simulink model "SVM_Stepper"  (R2020b)
settings: Solver=VariableStepAuto  StartTime=0.0  StopTime=1  FixedStep=0.0001  MaxStep=0.000005  RelTol=1e-3
values from neighbouring files (symbols this model uses):
  b = 0.05    [system_parameters.m]
  J = 48e-6    (= 4.8e-05)    [system_parameters.m]
  K_t = T_hold/I_rms    (= 0.575)    [system_parameters.m]
  L = 2e-3    (= 0.002)    [system_parameters.m]
  p = 50    [system_parameters.m]
  R = 0.5    [system_parameters.m]
  T_dm = 0.068    [system_parameters.m]
  T_load = 5.06e-3    (= 0.00506)    [system_parameters.m]
  U = 24    [system_parameters.m]
undefined symbols (not defined in the file or in its folder): Down, Up
libraries: fl_lib x90, ee_lib x55, eePwmGenerator x37, nesl_utility x33, dspsrcs4 x18, pid_lib x6, powerlib x4, eeDcCurrentController x1, eePmsmTorqueEstimator x1, simulink x1, eeQuadratureDecoder x1
(part 1 of 2)
settings Model: Creator=ginoa  LastModifiedBy=ginoa

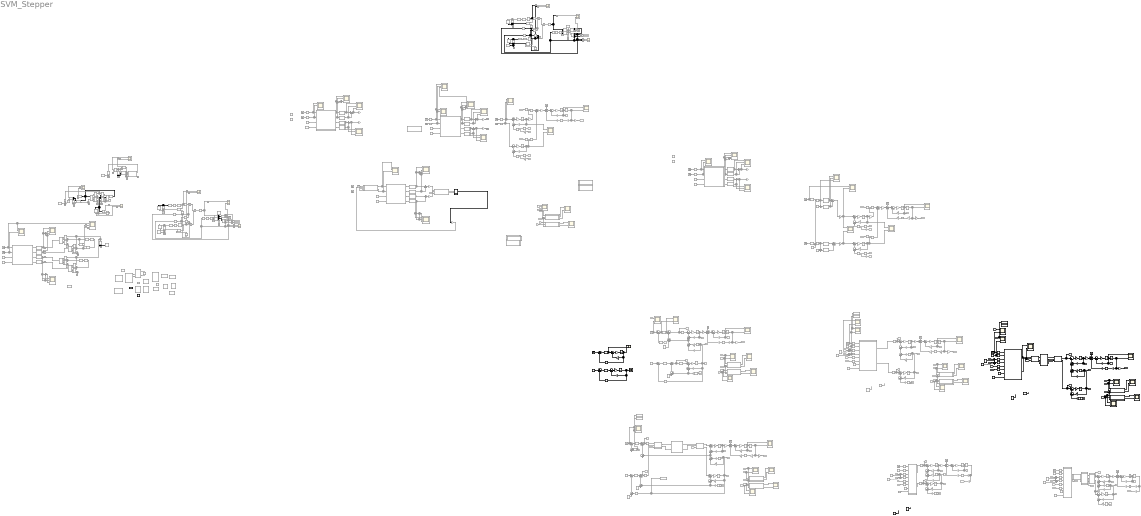
== system SVM_Stepper ==
  note: Load Torque
  note: Load Torque
  note: i_q
  note: i_d
  note: i_d
  note: i_q
  note: i_q
  note: i_d
  note: i_q
  note: i_d
  note: i_q
  note: i_d
  note: i_q
  note: i_d
  note: i_q
  note: i_d
  CMOS NOT : ee_lib/Integrated Circuits/Logic/CMOS NOT  Commented=on  V_IL=2 V  V_IH=3 V  C_IN=5 pF  output_type=1  V_OL=0 V  V_OH=5 V  V_CC=5 V  V_meas=5 V  R_OUT=25 Ohm  R_OH=[25, 250] Ohm  I_OH=63 mA  R_OL=[30, 800] Ohm  I_OL=-45 mA  Delay=25 ns  Ron=5 Ohm  Vf=0.6 V  output_state=1
      settings: SourceProductBaseCode=PS  InternalSimscapePortConfiguration="{\"Bottom\":[],\"Left\":[{\"id\":\"A\",\"label\":\"\",\"type\":\"foundation.electrical.electrical\"}],\"Right\":[{\"id\":\"J\",\"label\":\"\",\"type\":\"foundation.electrical.electrical\"}],\"Top\":[]}"
  Constant{,2,9,13,20,27,30} (7 alike) : Constant  Commented=on  Value=24
  Constant1 : Constant  Commented=on  Value=50e-6
  Constant10 : Constant  Commented=on  Value=48
  Constant11 : Constant  Commented=on  Value=25e-6
  Constant12 : Constant  Commented=on  Value=10
  Constant14 : Constant  Commented=on
  Constant15 : Constant  Commented=on  Value=48
  Constant16 : Constant  Commented=on
  Constant{17,19,22,26,29} (5 alike) : Constant  Commented=on  Value=0
  Constant18 : Constant  Value=0
  Constant21 : Constant  Commented=on  Value=20e-6
  Constant23 : Constant  Value=0
  Constant24 : Constant  Value=24
  Constant25 : Constant  Value=50e-6
  Constant28 : Constant  Commented=on  Value=50e-6
  Constant3 : Constant  Commented=on  Value=50e-6
  Constant31 : Constant  Commented=on  Value=20e-6
  Constant4 : Constant  Commented=on  Value=100
  Constant5 : Constant  Commented=on  Value=25e-6
  Constant6 : Constant  Commented=on  Value=48
  Constant7 : Constant  Commented=on  Value=25e-6
  Constant8 : Constant  Commented=on  Value=10
  Controlled PWM Voltage : ee_lib/Integrated Circuits/Controlled PWM Voltage  Commented=on  F=20000 Hz  TD=0 s  pulse_width_offset=0 s  pulse_min=0 s  Vmin=-24 V  Vmax=24 V  Vm=5 V  pwm_or_av=1  event_type=1  sample_time=1e-6 s  u_min=0  u_max=1
  Controlled PWM Voltage1 : ee_lib/Integrated Circuits/Controlled PWM Voltage  Commented=on  F=10000 Hz  TD=0 us  pulse_width_offset=0 s  pulse_min=4 us  Vmin=-24 V  Vmax=24 V  Vm=18 V  pwm_or_av=1  event_type=1  sample_time=1e-6 s  u_min=0  u_max=1
  Controlled PWM Voltage2 : ee_lib/Integrated Circuits/Controlled PWM Voltage  Commented=on  F=1000 Hz  TD=0 s  pulse_width_offset=0 s  pulse_min=0 s  Vmin=0 V  Vmax=5 V  Vm=5 V  pwm_or_av=1  event_type=1  sample_time=1e-6 s  u_min=0  u_max=1
  Controlled Voltage Source{,1..3} (4 alike) : fl_lib/Electrical/Electrical Sources/Controlled Voltage Source  Commented=on
  Cos{,1..3} (4 alike) : Trigonometry  Commented=on  Operator=cos
  Current Sensor{,1..5} (6 alike) : fl_lib/Electrical/Electrical Sensors/Current Sensor  Commented=on
  DC Current Controller : eeDcCurrentController/DC Current Controller  Commented=on  Kp=1  Ki=5  Kaw=1  VoltLim=Positive and negative voltage  Ts=-1  Tsd=0.001  ActZC=off
      settings: SourceProductBaseCode=PS
  DC Voltage Source : powerlib/Electrical Sources/DC Voltage Source  Commented=on  Amplitude=100  Measurements=None
  Deadbeat Control : MATLAB Function  TreatAsAtomicUnit=on
  Deadbeat Control1 : MATLAB Function  Commented=on  TreatAsAtomicUnit=on
  Divide : Product  Commented=on  Inputs=*/
  Divide1 : Product  Commented=on  Inputs=*/
  Electrical Reference{,1..21} (22 alike) : fl_lib/Electrical/Electrical Elements/Electrical Reference  Commented=on
  FCS MPC : MATLAB Function  Commented=on  TreatAsAtomicUnit=on
  FCS MPC1 : MATLAB Function  Commented=on  TreatAsAtomicUnit=on
  From{,4,22,30,45,77,86} (7 alike) : From  Commented=on  GotoTag=i_d
  From{1..3,23,26,31,34,38,44,46,49,53,72,76,80} (15 alike) : From  Commented=on  GotoTag=i_q
  From{5,8..11,13,15..17,19,21,27,35,41,50,54..55,79,82..83,88} (21 alike) : From  Commented=on  GotoTag=theta_e
  From{12,14,18,20,24..25,32..33,40,42..43,47..48,74..75,78,87} (17 alike) : From  Commented=on  GotoTag=w_m
  From{6,28,36,51} (4 alike) : From  Commented=on  GotoTag=u_q
  From{7,29,37,52} (4 alike) : From  Commented=on  GotoTag=u_d
  Full-Bridge Converter : powerlib/Power Electronics/Full-Bridge Converter  Commented=on  ModelType=Switching devices  Ron=1e-3  Rs=1e6  Cs=inf  Vforward=[0,0]  Ron_Diode=1e-3  Rs_Diode=1e6  Cs_Diode=inf  Vf_Diode=1e-3  Rs_CurrentSource=inf
      settings: SourceProductBaseCode=PS
  Gain{1,6,22,25,31,41,44,47,57,62,74,79,87,92,114,119} (16 alike) : Gain  Commented=on  Gain=K_t
  Gain{5,10,53,61,70,78,83,91,110,118} (10 alike) : Gain  Commented=on  Gain=L*p
  Gain100 : Gain  Gain=K_t
  Gain{64..65,101,103} (4 alike) : Gain  Gain=1/L
  Gain{63,66,95,102} (4 alike) : Gain  Gain=R
  Gain104 : Gain  Gain=L*p
  Gain105 : Gain  Gain=K_t
  Gain{20,39,56,73,86,106,113} (7 alike) : Gain  Commented=on  Gain=2*p
  Gain{7,16,35,50,67,80,107} (7 alike) : Gain  Commented=on  Gain=1/J
  Gain{8,17,36,51,68,81,108} (7 alike) : Gain  Commented=on  Gain=b
  Gain{3,9,24,30,43,46,52,59,69,76,82,89,109,116} (14 alike) : Gain  Commented=on  Gain=R
  Gain{11,18,37,54,71,84,111} (7 alike) : Gain  Commented=on  Gain=p
  Gain{13,19,38,55,72,85,112} (7 alike) : Gain  Commented=on  Gain=T_dm
  Gain{2,4,23,29,42,45,58,60,75,77,88,90,115,117} (14 alike) : Gain  Commented=on  Gain=1/L
  Gain12 : Gain  Commented=on  Gain=-1
  Gain{14..15,48..49} (4 alike) : Gain  Commented=on  Gain=24
  Gain21 : Gain  Commented=on  Gain=-1
  Gain26 : Gain  Commented=on  Gain=100
  Gain27 : Gain  Commented=on  Gain=100
  Gain{28,32..34} (4 alike) : Gain  Commented=on  Gain=48
  Gain40 : Gain  Commented=on  Gain=-1
  Gain93 : Gain  Gain=1/J
  Gain94 : Gain  Gain=b
  Gain96 : Gain  Gain=L*p
  Gain97 : Gain  Gain=p
  Gain98 : Gain  Gain=T_dm
  Gain99 : Gain  Gain=2*p
  Goto{1,14,20,26,39} (5 alike) : Goto  Commented=on  GotoTag=i_d
  Goto10 : Goto  Commented=on  GotoTag=PS_omega_m
  Goto11 : Goto  Commented=on  GotoTag=PS_theta_m
  Goto{3,8,12,16,22,28,41} (7 alike) : Goto  Commented=on  GotoTag=w_m
  Goto{6,9,13,17,23,29,42} (7 alike) : Goto  Commented=on  GotoTag=theta_e
  Goto{2,15,21,27,40} (5 alike) : Goto  Commented=on  GotoTag=i_q
  Goto{7,18,24,30,43} (5 alike) : Goto  Commented=on  GotoTag=u_q
  Goto{19,25,31,38,44} (5 alike) : Goto  Commented=on  GotoTag=u_d
  Goto4 : Goto  Commented=on  GotoTag=PS_omega_m
  Goto5 : Goto  Commented=on  GotoTag=PS_theta_m
  H-Bridge : ee_lib/Semiconductors & Converters/Converters/H-Bridge  Commented=on  supply_ports=ee.enum.supply_ports.hidesupply  Venable=2.5 V  Vmax=5.0 V  Vreverse=2.5 V  Vbrake=2.5 V  Vm=12 V  pwm_or_av=ee.enum.pwm_or_av.pwm  regenerative_braking_mode=ee.enum.converters.regenerative_braking_mode.depends_on_rev  discontinuous=ee.enum.current_profile.continuous  freewheeling_mode=ee.enum.converters.freewheeling_mode.one_switch_one_diode  Ron=0.1 Ohm  Don=0.05 Ohm  Goff=1e-6 S  Rload=10 Ohm  Lload=1e-5 H  F=10 kHz  thermal_mass=100 J/K  initial_temperature=298.15 K  Ron2=0.1 Ohm  Don2=0.05 Ohm  Tmeas=298.15 K  Tmeas2=398.15 K
  H-Bridge1 : ee_lib/Semiconductors & Converters/Converters/H-Bridge  Commented=on  supply_ports=ee.enum.supply_ports.hidesupply  Venable=2.5 V  Vmax=5.0 V  Vreverse=2.5 V  Vbrake=2.5 V  Vm=12 V  pwm_or_av=ee.enum.pwm_or_av.pwm  regenerative_braking_mode=ee.enum.converters.regenerative_braking_mode.depends_on_rev  discontinuous=ee.enum.current_profile.continuous  freewheeling_mode=ee.enum.converters.freewheeling_mode.one_switch_one_diode  Ron=0.1 Ohm  Don=0.05 Ohm  Goff=1e-6 S  Rload=10 Ohm  Lload=1e-5 H  F=10 kHz  thermal_mass=100 J/K  initial_temperature=298.15 K  Ron2=0.1 Ohm  Don2=0.05 Ohm  Tmeas=298.15 K  Tmeas2=398.15 K
  H-Bridge2 : ee_lib/Semiconductors & Converters/Converters/H-Bridge  Commented=on  supply_ports=ee.enum.supply_ports.showsupply  Venable=2.5 V  Vmax=5.0 V  Vreverse=2.5 V  Vbrake=2.5 V  Vm=12 V  pwm_or_av=ee.enum.pwm_or_av.pwm  regenerative_braking_mode=ee.enum.converters.regenerative_braking_mode.depends_on_rev  discontinuous=ee.enum.current_profile.continuous  freewheeling_mode=ee.enum.converters.freewheeling_mode.one_switch_one_diode  Ron=0.05 Ohm  Don=0.05 Ohm  Goff=1e-6 S  Rload=10 Ohm  Lload=1e-5 H  F=10 kHz  thermal_mass=100 J/K  initial_temperature=298.15 K  Ron2=0.1 Ohm  Don2=0.05 Ohm  Tmeas=298.15 K  Tmeas2=398.15 K
      settings: InternalSimscapePortConfiguration="{\"Bottom\":[],\"Left\":[{\"id\":\"ENA\",\"label\":\"PWM\",\"type\":\"foundation.electrical.electrical\"},{\"id\":\"REF\",\"label\":\"REF\",\"type\":\"foundation.electrical.electrical\"},{\"id\":\"REV\",\"label\":\"REV\",\"type\":\"foundation.electrical.electrical\"},{\"id\":\"BRK\",\"label\":\"BRK\",\"type\":\"foundation.electrical.electrical\"}],\"Right\":[{\"id\":\"p1\",\"label\":\"V+\",\"type\":\"foundation.electrical.electrical\"},{\"id\":\"p2\",\"label\":\"+\",\"type\":\"foundation.electrical.electrical\"},{\"id\":\"n2\",\"label\":\"-\",\"type\":\"foundation.electrical.electrical\"},{\"id\":\"n1\",\"label\":\"V-\",\"type\":\"foundation.electrical.electrical\"}],\"Top\":[]}"
  Half-Bridge Driver{,1..5} (6 alike) : ee_lib/Semiconductors & Converters/Half-Bridge Driver  Commented=on  vHigh=15 V  vLow=0 V  parameterization=1  rHigh=2 Ohm  rLow=2 Ohm  tRise=20 ns  tFall=20 ns  cLoad=10 nF  enable_faults=0  t_fault=1 s  fault_type=1  uHighValue=0.7  uLowValue=0.3  tpLH=50 ns  tdLH=100 ns  tpHL=50 ns  tdHL=100 ns  ZonTime_specify=off  ZonTime_priority=None  ZonTime=0 s  ZoffTime_specify=off  ZoffTime_priority=None  ZoffTime=0 s  power_dissipated_high_side_specify=off  power_dissipated_high_side_priority=None  power_dissipated_high_side=0 W  power_dissipated_high_side_nominal_specify=off  power_dissipated_high_side_nominal_unit=W  power_dissipated_high_side_nominal_value=1  power_dissipated_low_side_specify=off  power_dissipated_low_side_priority=None  power_dissipated_low_side=0 W  power_dissipated_low_side_nominal_specify=off  power_dissipated_low_side_nominal_unit=W  power_dissipated_low_side_nominal_value=1  uHigh=2.0 V  uLow=0.8 V
      Half-Bridge Driver settings: SourceProductBaseCode=PS  InternalSimscapePortConfiguration="{\"Bottom\":[],\"Left\":[{\"id\":\"PWM\",\"label\":\"PWM\",\"type\":\"foundation.electrical.electrical\"},{\"id\":\"REF\",\"label\":\"REF\",\"type\":\"foundation.electrical.electrical\"}],\"Right\":[{\"id\":\"HO\",\"label\":\"HO\",\"type\":\"foundation.electrical.electrical\"},{\"id\":\"HS\",\"label\":\"HS\",\"type\":\"foundation.electrical.electrical\"},{\"id\":\"LO\",\"label\":\"LO\",\"type\":\"foundation.electrical.electrical\"},{\"id\":\"LS\",\"label\":\"LS\",\"type\":\"foundation.electrical.electrical\"}],\"Top\":[]}"
      Half-Bridge Driver1 settings: SourceProductBaseCode=PS  InternalSimscapePortConfiguration="{\"Bottom\":[],\"Left\":[{\"id\":\"PWM\",\"label\":\"PWM\",\"type\":\"foundation.electrical.electrical\"},{\"id\":\"REF\",\"label\":\"REF\",\"type\":\"foundation.electrical.electrical\"}],\"Right\":[{\"id\":\"HO\",\"label\":\"HO\",\"type\":\"foundation.electrical.electrical\"},{\"id\":\"HS\",\"label\":\"HS\",\"type\":\"foundation.electrical.electrical\"},{\"id\":\"LO\",\"label\":\"LO\",\"type\":\"foundation.electrical.electrical\"},{\"id\":\"LS\",\"label\":\"LS\",\"type\":\"foundation.electrical.electrical\"}],\"Top\":[]}"
      Half-Bridge Driver2 settings: SourceProductBaseCode=PS  InternalSimscapePortConfiguration="{\"Bottom\":[],\"Left\":[{\"id\":\"u\",\"label\":\"u\",\"type\":\"input\"}],\"Right\":[{\"id\":\"HO\",\"label\":\"HO\",\"type\":\"foundation.electrical.electrical\"},{\"id\":\"HS\",\"label\":\"HS\",\"type\":\"foundation.electrical.electrical\"},{\"id\":\"LO\",\"label\":\"LO\",\"type\":\"foundation.electrical.electrical\"},{\"id\":\"LS\",\"label\":\"LS\",\"type\":\"foundation.electrical.electrical\"}],\"Top\":[]}"
      Half-Bridge Driver3 settings: SourceProductBaseCode=PS  InternalSimscapePortConfiguration="{\"Bottom\":[],\"Left\":[{\"id\":\"u\",\"label\":\"u\",\"type\":\"input\"}],\"Right\":[{\"id\":\"HO\",\"label\":\"HO\",\"type\":\"foundation.electrical.electrical\"},{\"id\":\"HS\",\"label\":\"HS\",\"type\":\"foundation.electrical.electrical\"},{\"id\":\"LO\",\"label\":\"LO\",\"type\":\"foundation.electrical.electrical\"},{\"id\":\"LS\",\"label\":\"LS\",\"type\":\"foundation.electrical.electrical\"}],\"Top\":[]}"
      Half-Bridge Driver4 settings: SourceProductBaseCode=PS  InternalSimscapePortConfiguration="{\"Bottom\":[],\"Left\":[{\"id\":\"u\",\"label\":\"u\",\"type\":\"input\"}],\"Right\":[{\"id\":\"HO\",\"label\":\"HO\",\"type\":\"foundation.electrical.electrical\"},{\"id\":\"HS\",\"label\":\"HS\",\"type\":\"foundation.electrical.electrical\"},{\"id\":\"LO\",\"label\":\"LO\",\"type\":\"foundation.electrical.electrical\"},{\"id\":\"LS\",\"label\":\"LS\",\"type\":\"foundation.electrical.electrical\"}],\"Top\":[]}"
      Half-Bridge Driver5 settings: SourceProductBaseCode=PS  InternalSimscapePortConfiguration="{\"Bottom\":[],\"Left\":[{\"id\":\"u\",\"label\":\"u\",\"type\":\"input\"}],\"Right\":[{\"id\":\"HO\",\"label\":\"HO\",\"type\":\"foundation.electrical.electrical\"},{\"id\":\"HS\",\"label\":\"HS\",\"type\":\"foundation.electrical.electrical\"},{\"id\":\"LO\",\"label\":\"LO\",\"type\":\"foundation.electrical.electrical\"},{\"id\":\"LS\",\"label\":\"LS\",\"type\":\"foundation.electrical.electrical\"}],\"Top\":[]}"
  Ideal Rotational Motion Sensor : fl_lib/Mechanical/Mechanical Sensors/Ideal Rotational Motion Sensor  Commented=on  wrap_angle=simscape.enum.onoff.off  offset=0 rad
  Ideal Rotational Motion Sensor1 : fl_lib/Mechanical/Mechanical Sensors/Ideal Rotational Motion Sensor  Commented=on  wrap_angle=simscape.enum.onoff.off  offset=0 rad
  Ideal Semiconductor Switch{,1..11} (12 alike) : ee_lib/Semiconductors & Converters/Ideal Semiconductor Switch  Commented=on  Ron=0.001 Ohm  Goff=1e-6 1/Ohm  Vth=0.5 V  diode_param=2  diode_Vf=0.8 V  diode_Ron=0.001 Ohm  diode_Goff=1e-5 1/Ohm  diode_C=50e-9 F  diode_iRM=-235 A  diode_iF=300 A  diode_idot=-50 A/us  diode_trr_param=1  diode_trr_factor=3  diode_trr=15 us  diode_Qrr=1500 s*uA
      settings: SourceProductBaseCode=PS  InternalSimscapePortConfiguration="{\"Bottom\":[],\"Left\":[{\"id\":\"G\",\"label\":\"\",\"type\":\"foundation.electrical.electrical\"}],\"Right\":[{\"id\":\"A\",\"label\":\"a\",\"type\":\"foundation.electrical.electrical\"},{\"id\":\"K\",\"label\":\"k\",\"type\":\"foundation.electrical.electrical\"}],\"Top\":[]}"
  Ideal Torque Source{,1..5} (6 alike) : fl_lib/Mechanical/Mechanical Sources/Ideal Torque Source  Commented=on
  Incremental Shaft Encoder : ee_lib/Sensors & Transducers/Incremental Shaft Encoder  Commented=on  NPulse=2  Vm=5 V  angle0=0 deg
      settings: SourceProductBaseCode=PS  InternalSimscapePortConfiguration="{\"Bottom\":[],\"Left\":[{\"id\":\"R\",\"label\":\"R\",\"type\":\"foundation.mechanical.rotational.rotational\"},{\"id\":\"C\",\"label\":\"C\",\"type\":\"foundation.mechanical.rotational.rotational\"}],\"Right\":[{\"id\":\"A\",\"label\":\"A\",\"type\":\"foundation.electrical.electrical\"},{\"id\":\"B\",\"label\":\"B\",\"type\":\"foundation.electrical.electrical\"},{\"id\":\"Z\",\"label\":\"Z\",\"type\":\"foundation.electrical.electrical\"},{\"id\":\"GND\",\"label\":\"REF\",\"type\":\"foundation.electrical.electrical\"}],\"Top\":[]}"
  Inductor{,1..2,4..6} (6 alike) : ee_lib/Passive/Inductor  Commented=on  l=L H  L_tol=20  enable_L_tol=0  tol_distribution=1  nSigma=4  r=0 Ohm  g=1e-9 1/Ohm  enable_operating_limits=0  operating_limit_action=2  max_working_current=1 A  power_rating=1 W  enable_faults=0  fault_action=1  lambdaPercent=50  k_faulted=0.9999  turnsShort=0  openCct=0  groundShort=0  groundShortG=0 1/Ohm  tau_fault=1e-3 s  enable_temporal_fault=0  t_fault=1 s  enable_behavioral_fault=0  max_permissible_voltage=100 V  n_fail_on_voltage=1  max_permissible_current=1 A  t_fail_on_current=1 s  i_L_specify=off  i_L_priority=High  i_L=0 A  i_L_nominal_specify=off  i_L_nominal_unit=A  i_L_nominal_value=1
  Inductor3 : ee_lib/Passive/Inductor  Commented=on  l=20 mH  L_tol=20  enable_L_tol=0  tol_distribution=1  nSigma=4  r=0 Ohm  g=1e-9 1/Ohm  enable_operating_limits=0  operating_limit_action=2  max_working_current=1 A  power_rating=1 W  enable_faults=0  fault_action=1  lambdaPercent=50  k_faulted=0.9999  turnsShort=0  openCct=0  groundShort=0  groundShortG=0 1/Ohm  tau_fault=1e-3 s  enable_temporal_fault=0  t_fault=1 s  enable_behavioral_fault=0  max_permissible_voltage=100 V  n_fail_on_voltage=1  max_permissible_current=1 A  t_fail_on_current=1 s  i_L_specify=off  i_L_priority=High  i_L=0 A  i_L_nominal_specify=off  i_L_nominal_unit=A  i_L_nominal_value=1
  Inertia : fl_lib/Mechanical/Rotational Elements/Inertia  Commented=on  inertia=J kg*m^2  num_ports=foundation.enum.numPorts2.one  w_specify=off  w_priority=High  w=0 rad/s  w_nominal_specify=off  w_nominal_unit=rad/s  w_nominal_value=1  t_specify=off  t_priority=None  t=0 N*m  t_nominal_specify=off  t_nominal_unit=N*m  t_nominal_value=1
  Inertia1 : fl_lib/Mechanical/Rotational Elements/Inertia  Commented=on  inertia=J kg*m^2  num_ports=foundation.enum.numPorts2.one  w_specify=off  w_priority=High  w=0 rad/s  w_nominal_specify=off  w_nominal_unit=rad/s  w_nominal_value=1  t_specify=off  t_priority=None  t=0 N*m  t_nominal_specify=off  t_nominal_unit=N*m  t_nominal_value=1
  Integrator{1..15,18..25,30..34} (28 alike) : Integrator  Commented=on
  Integrator16 : Integrator  InitialCondition=0.25
  Integrator{17,26..29} (5 alike) : Integrator
  MATLAB Function : MATLAB Function  Commented=on  TreatAsAtomicUnit=on
  MATLAB Function1 : MATLAB Function  Commented=on  TreatAsAtomicUnit=on
  MATLAB Function10 : MATLAB Function  Commented=on  TreatAsAtomicUnit=on
  MATLAB Function11 : MATLAB Function  Commented=on  TreatAsAtomicUnit=on
  MATLAB Function12 : MATLAB Function  Commented=on  TreatAsAtomicUnit=on
  MATLAB Function13 : MATLAB Function  Commented=on  TreatAsAtomicUnit=on
  MATLAB Function14 : MATLAB Function  Commented=on  TreatAsAtomicUnit=on
  MATLAB Function15 : MATLAB Function  Commented=on  TreatAsAtomicUnit=on
  MATLAB Function16 : MATLAB Function  Commented=on  TreatAsAtomicUnit=on
  MATLAB Function17 : MATLAB Function  Commented=on  TreatAsAtomicUnit=on
  MATLAB Function18 : MATLAB Function  TreatAsAtomicUnit=on
  MATLAB Function19 : MATLAB Function  TreatAsAtomicUnit=on
  MATLAB Function2 : MATLAB Function  Commented=on  TreatAsAtomicUnit=on
  MATLAB Function20 : MATLAB Function  TreatAsAtomicUnit=on
  MATLAB Function21 : MATLAB Function  TreatAsAtomicUnit=on
  MATLAB Function24 : MATLAB Function  Commented=on  TreatAsAtomicUnit=on
  MATLAB Function25 : MATLAB Function  Commented=on  TreatAsAtomicUnit=on
  MATLAB Function3 : MATLAB Function  Commented=on  TreatAsAtomicUnit=on
  MATLAB Function4 : MATLAB Function  Commented=on  TreatAsAtomicUnit=on
  MATLAB Function5 : MATLAB Function  Commented=on  TreatAsAtomicUnit=on
  MATLAB Function6 : MATLAB Function  Commented=on  TreatAsAtomicUnit=on
  MATLAB Function7 : MATLAB Function  Commented=on  TreatAsAtomicUnit=on
  MATLAB Function8 : MATLAB Function  Commented=on  TreatAsAtomicUnit=on
  MATLAB Function9 : MATLAB Function  Commented=on  TreatAsAtomicUnit=on
  Mechanical Rotational Reference{,1..5} (6 alike) : fl_lib/Mechanical/Rotational Elements/Mechanical Rotational Reference  Commented=on
  Modulator : Subsystem  Commented=on
  Modulator1 : Subsystem
  Modulator2 : Subsystem  Commented=on
  PID Controller1 : pid_lib/PID Controller  Controller=PI  Form=Parallel  TimeDomain=Discrete-time  UseExternalTs=off  SampleTime=50e-6  IntegratorMethod=Forward Euler  FilterMethod=Forward Euler  ControllerParametersSource=internal  P=2.70016858796685  I=1625.58138019351  D=0  UseFilter=on  N=100  TunerSelectOption=Transfer Function Based (PID Tuner App)  InitialConditionSource=internal  InitialConditionForIntegrator=0  InitialConditionForFilter=0  DifferentiatorICPrevScaledInput=0  ExternalReset=none  TrackingMode=off  Kt=1  LimitOutput=off  SatLimitsSource=external  UpperSaturationLimit=inf  LowerSaturationLimit=-inf  LinearizeAsGain=on  AntiWindupMode=none  Kb=1  POutMin=[]  POutMax=[]  IOutMin=[]  IOutMax=[]  DOutMin=[]  DOutMax=[]  NOutMin=[]  NOutMax=[]  SumOutMin=[]  SumOutMax=[]  SaturationOutMin=[]  SaturationOutMax=[]  PParamMin=[]  PParamMax=[]  IParamMin=[]  IParamMax=[]  DParamMin=[]  DParamMax=[]  NParamMin=[]  NParamMax=[]  KbParamMin=[]  KbParamMax=[]  KtParamMin=[]  KtParamMax=[]  KbOutMin=[]  KbOutMax=[]  KtOutMin=[]  KtOutMax=[]  IntegratorOutMin=[]  IntegratorOutMax=[]  FilterOutMin=[]  FilterOutMax=[]  SumI1OutMin=[]  SumI1OutMax=[]  SumI2OutMin=[]  SumI2OutMax=[]  SumI3OutMin=[]  SumI3OutMax=[]  SumI4OutMin=[]  SumI4OutMax=[]  SumDOutMin=[]  SumDOutMax=[]  DifferentiatorOutMin=[]  DifferentiatorOutMax=[]  FilterDiffOutCoefMin=[]  FilterDiffOutCoefMax=[]  ReciprocalOutMin=[]  ReciprocalOutMax=[]  SumDenOutMin=[]  SumDenOutMax=[]  SumNumOutMin=[]  SumNumOutMax=[]  DivideOutMin=[]  DivideOutMax=[]  UdiffTsProdOutMin=[]  UdiffTsProdOutMax=[]  NTsProdOutMin=[]  NTsProdOutMax=[]  UintegralTsProdOutMin=[]  UintegralTsProdOutMax=[]  UngainTsProdOutMin=[]  UngainTsProdOutMax=[]  IntegratorContinuousStateAttributes=''  IntegratorStateMustResolveToSignalObject=off  IntegratorRTWStateStorageClass=Auto  FilterContinuousStateAttributes=''  FilterStateMustResolveToSignalObject=off  FilterRTWStateStorageClass=Auto  ParallelPVariant=InternalParameters  IdealPVariant=Disabled  IVariant=InternalParameters  DVariant=Disabled  IntegratorVariant=Discrete  SatVariant=Disabled  AWVariant=Passthrough  PCopyVariant=Disabled  TRVariant=Disabled  FdbkBlocksVariant=Forward  IdealPFdbkVariant=Disabled  SatFdbkVariant=Disabled  DerivativeFilterVariant=Disabled  NVariant=Disabled  NCopyVariant=Disabled_SignalSpec  FilterICVariant=Disabled  IntegratorICVariant=InternalICs  ExternalResetVariant=Disabled  TRSumVariant=Passthrough  SumFdbkVariant=Disabled  SumVariant=Sum_PI  TsampFilterVariant=InternalTs  TsampNgainVariant=Passthrough  TsampIntegralVariant=Passthrough  ExternalSaturationOutDataTypeStr=Inherit: Same as second input
  PID Controller2 : pid_lib/PID Controller  Controller=PI  Form=Parallel  TimeDomain=Discrete-time  UseExternalTs=off  SampleTime=50e-6  IntegratorMethod=Forward Euler  FilterMethod=Forward Euler  ControllerParametersSource=internal  P=2.80095656977241  I=1871.29720535788  D=0  UseFilter=on  N=100  TunerSelectOption=Transfer Function Based (PID Tuner App)  InitialConditionSource=internal  InitialConditionForIntegrator=0  InitialConditionForFilter=0  DifferentiatorICPrevScaledInput=0  ExternalReset=none  TrackingMode=off  Kt=1  LimitOutput=off  SatLimitsSource=internal  UpperSaturationLimit=inf  LowerSaturationLimit=-inf  LinearizeAsGain=on  AntiWindupMode=none  Kb=1  POutMin=[]  POutMax=[]  IOutMin=[]  IOutMax=[]  DOutMin=[]  DOutMax=[]  NOutMin=[]  NOutMax=[]  SumOutMin=[]  SumOutMax=[]  SaturationOutMin=[]  SaturationOutMax=[]  PParamMin=[]  PParamMax=[]  IParamMin=[]  IParamMax=[]  DParamMin=[]  DParamMax=[]  NParamMin=[]  NParamMax=[]  KbParamMin=[]  KbParamMax=[]  KtParamMin=[]  KtParamMax=[]  KbOutMin=[]  KbOutMax=[]  KtOutMin=[]  KtOutMax=[]  IntegratorOutMin=[]  IntegratorOutMax=[]  FilterOutMin=[]  FilterOutMax=[]  SumI1OutMin=[]  SumI1OutMax=[]  SumI2OutMin=[]  SumI2OutMax=[]  SumI3OutMin=[]  SumI3OutMax=[]  SumI4OutMin=[]  SumI4OutMax=[]  SumDOutMin=[]  SumDOutMax=[]  DifferentiatorOutMin=[]  DifferentiatorOutMax=[]  FilterDiffOutCoefMin=[]  FilterDiffOutCoefMax=[]  ReciprocalOutMin=[]  ReciprocalOutMax=[]  SumDenOutMin=[]  SumDenOutMax=[]  SumNumOutMin=[]  SumNumOutMax=[]  DivideOutMin=[]  DivideOutMax=[]  UdiffTsProdOutMin=[]  UdiffTsProdOutMax=[]  NTsProdOutMin=[]  NTsProdOutMax=[]  UintegralTsProdOutMin=[]  UintegralTsProdOutMax=[]  UngainTsProdOutMin=[]  UngainTsProdOutMax=[]  IntegratorContinuousStateAttributes=''  IntegratorStateMustResolveToSignalObject=off  IntegratorRTWStateStorageClass=Auto  FilterContinuousStateAttributes=''  FilterStateMustResolveToSignalObject=off  FilterRTWStateStorageClass=Auto  ParallelPVariant=InternalParameters  IdealPVariant=Disabled  IVariant=InternalParameters  DVariant=Disabled  IntegratorVariant=Discrete  SatVariant=Disabled  AWVariant=Passthrough  PCopyVariant=Disabled  TRVariant=Disabled  FdbkBlocksVariant=Forward  IdealPFdbkVariant=Disabled  SatFdbkVariant=Disabled  DerivativeFilterVariant=Disabled  NVariant=Disabled  NCopyVariant=Disabled_SignalSpec  FilterICVariant=Disabled  IntegratorICVariant=InternalICs  ExternalResetVariant=Disabled  TRSumVariant=Passthrough  SumFdbkVariant=Disabled  SumVariant=Sum_PI  TsampFilterVariant=InternalTs  TsampNgainVariant=Passthrough  TsampIntegralVariant=Passthrough  ExternalSaturationOutDataTypeStr=Inherit: Same as second input
  PID Controller3 : pid_lib/PID Controller  Commented=on  Controller=PI  Form=Parallel  TimeDomain=Discrete-time  UseExternalTs=off  SampleTime=50e-6  IntegratorMethod=Forward Euler  FilterMethod=Forward Euler  ControllerParametersSource=internal  P=2.80095656977241  I=1871.29720535788  D=0  UseFilter=on  N=100  TunerSelectOption=Transfer Function Based (PID Tuner App)  InitialConditionSource=internal  InitialConditionForIntegrator=0  InitialConditionForFilter=0  DifferentiatorICPrevScaledInput=0  ExternalReset=none  TrackingMode=off  Kt=1  LimitOutput=off  SatLimitsSource=internal  UpperSaturationLimit=inf  LowerSaturationLimit=-inf  LinearizeAsGain=on  AntiWindupMode=none  Kb=1  POutMin=[]  POutMax=[]  IOutMin=[]  IOutMax=[]  DOutMin=[]  DOutMax=[]  NOutMin=[]  NOutMax=[]  SumOutMin=[]  SumOutMax=[]  SaturationOutMin=[]  SaturationOutMax=[]  PParamMin=[]  PParamMax=[]  IParamMin=[]  IParamMax=[]  DParamMin=[]  DParamMax=[]  NParamMin=[]  NParamMax=[]  KbParamMin=[]  KbParamMax=[]  KtParamMin=[]  KtParamMax=[]  KbOutMin=[]  KbOutMax=[]  KtOutMin=[]  KtOutMax=[]  IntegratorOutMin=[]  IntegratorOutMax=[]  FilterOutMin=[]  FilterOutMax=[]  SumI1OutMin=[]  SumI1OutMax=[]  SumI2OutMin=[]  SumI2OutMax=[]  SumI3OutMin=[]  SumI3OutMax=[]  SumI4OutMin=[]  SumI4OutMax=[]  SumDOutMin=[]  SumDOutMax=[]  DifferentiatorOutMin=[]  DifferentiatorOutMax=[]  FilterDiffOutCoefMin=[]  FilterDiffOutCoefMax=[]  ReciprocalOutMin=[]  ReciprocalOutMax=[]  SumDenOutMin=[]  SumDenOutMax=[]  SumNumOutMin=[]  SumNumOutMax=[]  DivideOutMin=[]  DivideOutMax=[]  UdiffTsProdOutMin=[]  UdiffTsProdOutMax=[]  NTsProdOutMin=[]  NTsProdOutMax=[]  UintegralTsProdOutMin=[]  UintegralTsProdOutMax=[]  UngainTsProdOutMin=[]  UngainTsProdOutMax=[]  IntegratorContinuousStateAttributes=''  IntegratorStateMustResolveToSignalObject=off  IntegratorRTWStateStorageClass=Auto  FilterContinuousStateAttributes=''  FilterStateMustResolveToSignalObject=off  FilterRTWStateStorageClass=Auto  ParallelPVariant=InternalParameters  IdealPVariant=Disabled  IVariant=InternalParameters  DVariant=Disabled  IntegratorVariant=Discrete  SatVariant=Disabled  AWVariant=Passthrough  PCopyVariant=Disabled  TRVariant=Disabled  FdbkBlocksVariant=Forward  IdealPFdbkVariant=Disabled  SatFdbkVariant=Disabled  DerivativeFilterVariant=Disabled  NVariant=Disabled  NCopyVariant=Disabled_SignalSpec  FilterICVariant=Disabled  IntegratorICVariant=InternalICs  ExternalResetVariant=Disabled  TRSumVariant=Passthrough  SumFdbkVariant=Disabled  SumVariant=Sum_PI  TsampFilterVariant=InternalTs  TsampNgainVariant=Passthrough  TsampIntegralVariant=Passthrough  ExternalSaturationOutDataTypeStr=Inherit: Same as second input
  PID Controller4 : pid_lib/PID Controller  Commented=on  Controller=PI  Form=Parallel  TimeDomain=Discrete-time  UseExternalTs=off  SampleTime=50e-6  IntegratorMethod=Forward Euler  FilterMethod=Forward Euler  ControllerParametersSource=internal  P=2.70016858796685  I=1625.58138019351  D=0  UseFilter=on  N=100  TunerSelectOption=Transfer Function Based (PID Tuner App)  InitialConditionSource=internal  InitialConditionForIntegrator=0  InitialConditionForFilter=0  DifferentiatorICPrevScaledInput=0  ExternalReset=none  TrackingMode=off  Kt=1  LimitOutput=off  SatLimitsSource=external  UpperSaturationLimit=inf  LowerSaturationLimit=-inf  LinearizeAsGain=on  AntiWindupMode=none  Kb=1  POutMin=[]  POutMax=[]  IOutMin=[]  IOutMax=[]  DOutMin=[]  DOutMax=[]  NOutMin=[]  NOutMax=[]  SumOutMin=[]  SumOutMax=[]  SaturationOutMin=[]  SaturationOutMax=[]  PParamMin=[]  PParamMax=[]  IParamMin=[]  IParamMax=[]  DParamMin=[]  DParamMax=[]  NParamMin=[]  NParamMax=[]  KbParamMin=[]  KbParamMax=[]  KtParamMin=[]  KtParamMax=[]  KbOutMin=[]  KbOutMax=[]  KtOutMin=[]  KtOutMax=[]  IntegratorOutMin=[]  IntegratorOutMax=[]  FilterOutMin=[]  FilterOutMax=[]  SumI1OutMin=[]  SumI1OutMax=[]  SumI2OutMin=[]  SumI2OutMax=[]  SumI3OutMin=[]  SumI3OutMax=[]  SumI4OutMin=[]  SumI4OutMax=[]  SumDOutMin=[]  SumDOutMax=[]  DifferentiatorOutMin=[]  DifferentiatorOutMax=[]  FilterDiffOutCoefMin=[]  FilterDiffOutCoefMax=[]  ReciprocalOutMin=[]  ReciprocalOutMax=[]  SumDenOutMin=[]  SumDenOutMax=[]  SumNumOutMin=[]  SumNumOutMax=[]  DivideOutMin=[]  DivideOutMax=[]  UdiffTsProdOutMin=[]  UdiffTsProdOutMax=[]  NTsProdOutMin=[]  NTsProdOutMax=[]  UintegralTsProdOutMin=[]  UintegralTsProdOutMax=[]  UngainTsProdOutMin=[]  UngainTsProdOutMax=[]  IntegratorContinuousStateAttributes=''  IntegratorStateMustResolveToSignalObject=off  IntegratorRTWStateStorageClass=Auto  FilterContinuousStateAttributes=''  FilterStateMustResolveToSignalObject=off  FilterRTWStateStorageClass=Auto  ParallelPVariant=InternalParameters  IdealPVariant=Disabled  IVariant=InternalParameters  DVariant=Disabled  IntegratorVariant=Discrete  SatVariant=Disabled  AWVariant=Passthrough  PCopyVariant=Disabled  TRVariant=Disabled  FdbkBlocksVariant=Forward  IdealPFdbkVariant=Disabled  SatFdbkVariant=Disabled  DerivativeFilterVariant=Disabled  NVariant=Disabled  NCopyVariant=Disabled_SignalSpec  FilterICVariant=Disabled  IntegratorICVariant=InternalICs  ExternalResetVariant=Disabled  TRSumVariant=Passthrough  SumFdbkVariant=Disabled  SumVariant=Sum_PI  TsampFilterVariant=InternalTs  TsampNgainVariant=Passthrough  TsampIntegralVariant=Passthrough  ExternalSaturationOutDataTypeStr=Inherit: Same as second input
  PID Controller5 : pid_lib/PID Controller  Commented=on  Controller=PI  Form=Parallel  TimeDomain=Discrete-time  UseExternalTs=off  SampleTime=50e-6  IntegratorMethod=Forward Euler  FilterMethod=Forward Euler  ControllerParametersSource=internal  P=2.80095656977241  I=1871.29720535788  D=0  UseFilter=on  N=100  TunerSelectOption=Transfer Function Based (PID Tuner App)  InitialConditionSource=internal  InitialConditionForIntegrator=0  InitialConditionForFilter=0  DifferentiatorICPrevScaledInput=0  ExternalReset=none  TrackingMode=off  Kt=1  LimitOutput=on  SatLimitsSource=internal  UpperSaturationLimit=inf  LowerSaturationLimit=-inf  LinearizeAsGain=on  AntiWindupMode=clamping  Kb=1  POutMin=[]  POutMax=[]  IOutMin=[]  IOutMax=[]  DOutMin=[]  DOutMax=[]  NOutMin=[]  NOutMax=[]  SumOutMin=[]  SumOutMax=[]  SaturationOutMin=[]  SaturationOutMax=[]  PParamMin=[]  PParamMax=[]  IParamMin=[]  IParamMax=[]  DParamMin=[]  DParamMax=[]  NParamMin=[]  NParamMax=[]  KbParamMin=[]  KbParamMax=[]  KtParamMin=[]  KtParamMax=[]  KbOutMin=[]  KbOutMax=[]  KtOutMin=[]  KtOutMax=[]  IntegratorOutMin=[]  IntegratorOutMax=[]  FilterOutMin=[]  FilterOutMax=[]  SumI1OutMin=[]  SumI1OutMax=[]  SumI2OutMin=[]  SumI2OutMax=[]  SumI3OutMin=[]  SumI3OutMax=[]  SumI4OutMin=[]  SumI4OutMax=[]  SumDOutMin=[]  SumDOutMax=[]  DifferentiatorOutMin=[]  DifferentiatorOutMax=[]  FilterDiffOutCoefMin=[]  FilterDiffOutCoefMax=[]  ReciprocalOutMin=[]  ReciprocalOutMax=[]  SumDenOutMin=[]  SumDenOutMax=[]  SumNumOutMin=[]  SumNumOutMax=[]  DivideOutMin=[]  DivideOutMax=[]  UdiffTsProdOutMin=[]  UdiffTsProdOutMax=[]  NTsProdOutMin=[]  NTsProdOutMax=[]  UintegralTsProdOutMin=[]  UintegralTsProdOutMax=[]  UngainTsProdOutMin=[]  UngainTsProdOutMax=[]  IntegratorContinuousStateAttributes=''  IntegratorStateMustResolveToSignalObject=off  IntegratorRTWStateStorageClass=Auto  FilterContinuousStateAttributes=''  FilterStateMustResolveToSignalObject=off  FilterRTWStateStorageClass=Auto  ParallelPVariant=InternalParameters  IdealPVariant=Disabled  IVariant=InternalParameters  DVariant=Disabled  IntegratorVariant=Discrete  SatVariant=Enabled  AWVariant=DiscClampingParallel  PCopyVariant=Disabled  TRVariant=Disabled  FdbkBlocksVariant=Forward  IdealPFdbkVariant=Disabled  SatFdbkVariant=Disabled  DerivativeFilterVariant=Disabled  NVariant=Disabled  NCopyVariant=Disabled_SignalSpec  FilterICVariant=Disabled  IntegratorICVariant=InternalICs  ExternalResetVariant=Disabled  TRSumVariant=Passthrough  SumFdbkVariant=Disabled  SumVariant=Sum_PI  TsampFilterVariant=InternalTs  TsampNgainVariant=Passthrough  TsampIntegralVariant=Passthrough  ExternalSaturationOutDataTypeStr=Inherit: Same as second input
  PID Controller6 : pid_lib/PID Controller  Commented=on  Controller=PI  Form=Parallel  TimeDomain=Discrete-time  UseExternalTs=off  SampleTime=50e-6  IntegratorMethod=Forward Euler  FilterMethod=Forward Euler  ControllerParametersSource=internal  P=2.70016858796685  I=1625.58138019351  D=0  UseFilter=on  N=100  TunerSelectOption=Transfer Function Based (PID Tuner App)  InitialConditionSource=internal  InitialConditionForIntegrator=0  InitialConditionForFilter=0  DifferentiatorICPrevScaledInput=0  ExternalReset=none  TrackingMode=off  Kt=1  LimitOutput=on  SatLimitsSource=internal  UpperSaturationLimit=inf  LowerSaturationLimit=-inf  LinearizeAsGain=on  AntiWindupMode=clamping  Kb=1  POutMin=[]  POutMax=[]  IOutMin=[]  IOutMax=[]  DOutMin=[]  DOutMax=[]  NOutMin=[]  NOutMax=[]  SumOutMin=[]  SumOutMax=[]  SaturationOutMin=[]  SaturationOutMax=[]  PParamMin=[]  PParamMax=[]  IParamMin=[]  IParamMax=[]  DParamMin=[]  DParamMax=[]  NParamMin=[]  NParamMax=[]  KbParamMin=[]  KbParamMax=[]  KtParamMin=[]  KtParamMax=[]  KbOutMin=[]  KbOutMax=[]  KtOutMin=[]  KtOutMax=[]  IntegratorOutMin=[]  IntegratorOutMax=[]  FilterOutMin=[]  FilterOutMax=[]  SumI1OutMin=[]  SumI1OutMax=[]  SumI2OutMin=[]  SumI2OutMax=[]  SumI3OutMin=[]  SumI3OutMax=[]  SumI4OutMin=[]  SumI4OutMax=[]  SumDOutMin=[]  SumDOutMax=[]  DifferentiatorOutMin=[]  DifferentiatorOutMax=[]  FilterDiffOutCoefMin=[]  FilterDiffOutCoefMax=[]  ReciprocalOutMin=[]  ReciprocalOutMax=[]  SumDenOutMin=[]  SumDenOutMax=[]  SumNumOutMin=[]  SumNumOutMax=[]  DivideOutMin=[]  DivideOutMax=[]  UdiffTsProdOutMin=[]  UdiffTsProdOutMax=[]  NTsProdOutMin=[]  NTsProdOutMax=[]  UintegralTsProdOutMin=[]  UintegralTsProdOutMax=[]  UngainTsProdOutMin=[]  UngainTsProdOutMax=[]  IntegratorContinuousStateAttributes=''  IntegratorStateMustResolveToSignalObject=off  IntegratorRTWStateStorageClass=Auto  FilterContinuousStateAttributes=''  FilterStateMustResolveToSignalObject=off  FilterRTWStateStorageClass=Auto  ParallelPVariant=InternalParameters  IdealPVariant=Disabled  IVariant=InternalParameters  DVariant=Disabled  IntegratorVariant=Discrete  SatVariant=Enabled  AWVariant=DiscClampingParallel  PCopyVariant=Disabled  TRVariant=Disabled  FdbkBlocksVariant=Forward  IdealPFdbkVariant=Disabled  SatFdbkVariant=Disabled  DerivativeFilterVariant=Disabled  NVariant=Disabled  NCopyVariant=Disabled_SignalSpec  FilterICVariant=Disabled  IntegratorICVariant=InternalICs  ExternalResetVariant=Disabled  TRSumVariant=Passthrough  SumFdbkVariant=Disabled  SumVariant=Sum_PI  TsampFilterVariant=InternalTs  TsampNgainVariant=Passthrough  TsampIntegralVariant=Passthrough  ExternalSaturationOutDataTypeStr=Inherit: Same as second input
  PMSM : ee_lib/Electromechanical/Permanent Magnet/PMSM  Commented=on  winding_type=ee.enum.statorconnection.wye  machine_param=ee.enum.pmsm.parameterization.constant  nPolePairs=6  pmflux_param=ee.enum.pmflux.fluxlinkage  pm_flux_linkage=0.03 Wb  torque_constant=0.18 N*m/A  back_emf_constant=0.18 V/(rad/s)  stator_param=ee.enum.statorparam.LdLqL0  Ld=0.00019 H  Lq=0.00025 H  idVec=[-200, 0, 200] A  iqVec=[-200, 0, 200] A  LdMatrix=0.0002 * ones(3, 3) H  LqMatrix=0.0002 * ones(3, 3) H  PmMatrix=0.1 * ones(3, 3) Wb  ktMatrix=0.18 * ones(3, 3) N*m/A  keMatrix=0.18 * ones(3, 3) V/(rad/s)  L0=0.00016 H  Ls=0.0002 H  Lm=-0.00002 H  Ms=0.00002 H  Rs=0.013 Ohm  zero_sequence=ee.enum.park.zerosequence.include  J=0.01 kg*m^2  lam=0 N*m/(rad/s)  axes_param=ee.enum.rotorangle.daxis  i_d_specify=off  i_d_priority=None  i_d=0 A  i_d_nominal_specify=off  i_d_nominal_unit=A  i_d_nominal_value=1  i_q_specify=off  i_q_priority=None  i_q=0 A  i_q_nominal_specify=off  i_q_nominal_unit=A  i_q_nominal_value=1  torque_specify=off  torque_priority=None  torque=0 N*m  torque_nominal_specify=off  torque_nominal_unit=N*m  torque_nominal_value=1  angular_velocity_specify=off  angular_velocity_priority=High  angular_velocity=0 rpm  angular_velocity_nominal_specify=off  angular_velocity_nominal_unit=rpm  angular_velocity_nominal_value=1  angular_position_specify=off  angular_position_priority=High  angular_position=0 deg  angular_position_nominal_specify=off  angular_position_nominal_unit=deg  angular_position_nominal_value=1  loss_param=ee.enum.ironloss.none  losses_oc=[0, 0, 0] W  losses_sc=[0, 0, 0] W  f_losses=60 Hz  Isc_losses=95 A  Tmeas=298.15 K  alpha=3.93e-3 1/K  alpha_flux=-0.001 1/K  stator_thermal_mass=100 J/K  rotor_thermal_mass=200 J/K  Rm_percent_rotor=90  Rd_percent_rotor=30  temperatureA_specify=off  temperatureA_priority=High  temperatureA=25 degC  temperatureA_nominal_specify=off  temperatureA_nominal_unit=degC  temperatureA_nominal_value=1  temperatureB_specify=off  temperatureB_priority=High  temperatureB=25 degC  temperatureB_nominal_specify=off  temperatureB_nominal_unit=degC  temperatureB_nominal_value=1  temperatureC_specify=off  temperatureC_priority=High  temperatureC=25 degC  temperatureC_nominal_specify=off  temperatureC_nominal_unit=degC  temperatureC_nominal_value=1  temperatureR_specify=off  temperatureR_priority=High  temperatureR=25 degC  temperatureR_nominal_specify=off  temperatureR_nominal_unit=degC  temperatureR_nominal_value=1
      settings: InternalSimscapePortConfiguration="{\"Bottom\":[],\"Left\":[{\"id\":\"N\",\"label\":\"~\",\"type\":\"foundation.electrical.three_phase\"},{\"id\":\"n\",\"label\":\"n\",\"type\":\"foundation.electrical.electrical\"}],\"Right\":[{\"id\":\"R\",\"label\":\"R\",\"type\":\"foundation.mechanical.rotational.rotational\"},{\"id\":\"C\",\"label\":\"C\",\"type\":\"foundation.mechanical.rotational.rotational\"}],\"Top\":[]}"
  PMSM Torque Estimator : eePmsmTorqueEstimator/PMSM Torque Estimator  Commented=on  ParamType=Constant parameters  p=8  idVect=[-200, 200]  iqVect=[-200, 200]  LdMatrix=0.0002 * ones(2, 2)  LqMatrix=0.0002 * ones(2, 2)  psimMatrix=0.04 * ones(2, 2)  Ld=0.0002  Lq=0.0002  psim=0.04  Ts=-1
      settings: SourceProductBaseCode=PS
  PS Add : fl_lib/Physical Signals/Functions/PS Add  Commented=on
  PS Add1 : fl_lib/Physical Signals/Functions/PS Add  Commented=on
  PS Gain : fl_lib/Physical Signals/Functions/PS Gain  Commented=on  gain=-1
  PS Gain{1,5,7,11} (4 alike) : fl_lib/Physical Signals/Functions/PS Gain  Commented=on  gain=K_t N*m/A
  PS Gain10 : fl_lib/Physical Signals/Functions/PS Gain  Commented=on  gain=p
  PS Gain2 : fl_lib/Physical Signals/Functions/PS Gain  Commented=on  gain=2*p
  PS Gain3 : fl_lib/Physical Signals/Functions/PS Gain  Commented=on  gain=-T_dm N*m
  PS Gain4 : fl_lib/Physical Signals/Functions/PS Gain  Commented=on  gain=p
  PS Gain6 : fl_lib/Physical Signals/Functions/PS Gain  Commented=on  gain=-1
  PS Gain8 : fl_lib/Physical Signals/Functions/PS Gain  Commented=on  gain=2*p
  PS Gain9 : fl_lib/Physical Signals/Functions/PS Gain  Commented=on  gain=-T_dm N*m
  PS Math Function : fl_lib/Physical Signals/Functions/PS Math Function  Commented=on  fcn_choice=foundation.enum.math_function.cos
      settings: SourceProductBaseCode=SS
  PS Math Function{1,3..4,6} (4 alike) : fl_lib/Physical Signals/Functions/PS Math Function  Commented=on  fcn_choice=foundation.enum.math_function.sin
      settings: SourceProductBaseCode=SS
  PS Math Function2 : fl_lib/Physical Signals/Functions/PS Math Function  Commented=on  fcn_choice=foundation.enum.math_function.cos
      settings: SourceProductBaseCode=SS
  PS Math Function5 : fl_lib/Physical Signals/Functions/PS Math Function  Commented=on  fcn_choice=foundation.enum.math_function.cos
      settings: SourceProductBaseCode=SS
  PS Product{,1..7} (8 alike) : fl_lib/Physical Signals/Functions/PS Product  Commented=on
  PS-Simulink Converter{,1..21} (22 alike) : nesl_utility/PS-Simulink Converter  Commented=on  PhysicalDomain=network_engine_domain  SubClassName=ps_output  LeftPortType=input  RightPortType=output  PseudoPeriodic=off  Frequencies=[]  Unit=inherit  AffineConversion=off
  PWM : simulink/Discontinuities/PWM  Commented=on  DisableCoverage=on  Period=1  DisallowZeroDutyCycle=off  RunAtFixedTimeIntervals=off  SampleTime=0.1
  PWM Generator : eePwmGenerator/PWM Generator  Commented=on  CarrCount=Up  Tper=0.001  Ts=5e-5
  PWM Generator{1..8} (8 alike) : eePwmGenerator/PWM Generator  Commented=on  CarrCount=Up-Down  Tper=25e-6  Ts=1e-6
  PWM Generator{9..20} (12 alike) : eePwmGenerator/PWM Generator  Commented=on  CarrCount=Up-Down  Tper=12.5e-6  Ts=1e-6
  PWM Generator{21..24} (4 alike) : eePwmGenerator/PWM Generator  Commented=on  CarrCount=Up  Tper=25e-6  Ts=1e-6
  Product{1..15,18..20} (18 alike) : Product  Commented=on
  Product16 : Product
  Product17 : Product
  Programmable Voltage Source : ee_lib/Sources/Programmable Voltage Source  Commented=on  magnitude_type=ee.enum.timechanging.external  ac_magnitude=100 V  magn_ramp=1 V/s  magn_step=1 V  magn_modu_magn=1 V  magn_modu_freq=1 Hz  magn_t1=1 s  magn_t2=2 s  frequency_type=ee.enum.timechanging.constant  ac_frequency=60 Hz  freq_ramp=1 Hz/s  freq_step=1 Hz  freq_modu_magn=1 Hz  freq_modu_freq=1 Hz  freq_t1=1 s  freq_t2=2 s  phase_type=ee.enum.timechanging.constant  ac_shift=0 deg  phase_ramp=1 deg/s  phase_step=1 deg  phase_modu_magn=1 deg  phase_modu_freq=1 Hz  phase_t1=1 s  phase_t2=2 s  dc_type=ee.enum.timechanging.external  dc_voltage=0 V  dc_ramp=1 V/s  dc_step=1 V  dc_modu_magn=1 V  dc_modu_freq=1 Hz  dc_t1=1 s  dc_t2=2 s  harmonic_option=0  noise_mode=0  PSD=0 V^2/Hz  repeatability=1  auto_seed=0  user_seed=0  sample_time=1e-3 s  harmonic_orders=[5, 7, 11, 13]  harmonic_ratios=[.1, .1, .1, .1]  harmonic_shifts=[0, 0, 0, 0] deg  harmonic_t1=-inf s  harmonic_t2=inf s  i_specify=off  i_priority=None  i=0 A  i_nominal_specify=off  i_nominal_unit=A  i_nominal_value=1  v_specify=off  v_priority=None  v=0 V  v_nominal_specify=off  v_nominal_unit=V  v_nominal_value=1
      settings: SourceProductBaseCode=PS  InternalSimscapePortConfiguration="{\"Bottom\":[],\"Left\":[{\"id\":\"p\",\"label\":\"+\",\"type\":\"foundation.electrical.electrical\"}],\"Right\":[{\"id\":\"ext_dc\",\"label\":\"DC\",\"type\":\"input\"},{\"id\":\"ext_magn\",\"label\":\"M\",\"type\":\"input\"},{\"id\":\"n\",\"label\":\"-\",\"type\":\"foundation.electrical.electrical\"}],\"Top\":[]}"
  Quadrature Shaft Decoder : eeQuadratureDecoder/Quadrature Shaft Decoder  Commented=on  NPulse=4  Ts=-1
      settings: SourceProductBaseCode=PS
  Random Source{,1..4} (5 alike) : dspsrcs4/Random Source  Commented=on  SrcType=Uniform  NormMethod=Ziggurat  CltLength=12  MinVal=-0.05  MaxVal=0.05  MeanVal=0  VarVal=1  RepMode=Not repeatable  rawSeed=1  IsInherit=off  SampMode=Discrete  SampTime=.001  SampFrame=1  DataType=Double  OutComplex=Real  OutputFrames=off
  Random Source10 : dspsrcs4/Random Source  Commented=on  SrcType=Gaussian  NormMethod=Ziggurat  CltLength=12  MinVal=-0.01  MaxVal=0.01  MeanVal=0  VarVal=0.00005  RepMode=Not repeatable  rawSeed=1  IsInherit=off  SampMode=Discrete  SampTime=.001  SampFrame=1  DataType=Double  OutComplex=Real  OutputFrames=off
  Random Source11 : dspsrcs4/Random Source  Commented=on  SrcType=Gaussian  NormMethod=Ziggurat  CltLength=12  MinVal=-0.05  MaxVal=0.05  MeanVal=0  VarVal=0.00005  RepMode=Not repeatable  rawSeed=1  IsInherit=off  SampMode=Discrete  SampTime=.001  SampFrame=1  DataType=Double  OutComplex=Real  OutputFrames=off
  Random Source12 : dspsrcs4/Random Source  Commented=on  SrcType=Gaussian  NormMethod=Ziggurat  CltLength=12  MinVal=-0.01  MaxVal=0.01  MeanVal=0  VarVal=0.00005  RepMode=Not repeatable  rawSeed=1  IsInherit=off  SampMode=Discrete  SampTime=.001  SampFrame=1  DataType=Double  OutComplex=Real  OutputFrames=off
  Random Source13 : dspsrcs4/Random Source  Commented=on  SrcType=Gaussian  NormMethod=Ziggurat  CltLength=12  MinVal=-0.05  MaxVal=0.05  MeanVal=0  VarVal=0.00005  RepMode=Not repeatable  rawSeed=1  IsInherit=off  SampMode=Discrete  SampTime=.001  SampFrame=1  DataType=Double  OutComplex=Real  OutputFrames=off
  Random Source14 : dspsrcs4/Random Source  Commented=on  SrcType=Gaussian  NormMethod=Ziggurat  CltLength=12  MinVal=-0.01  MaxVal=0.01  MeanVal=0  VarVal=0.00025  RepMode=Not repeatable  rawSeed=1  IsInherit=off  SampMode=Discrete  SampTime=.001  SampFrame=1  DataType=Double  OutComplex=Real  OutputFrames=off
  Random Source15 : dspsrcs4/Random Source  Commented=on  SrcType=Gaussian  NormMethod=Ziggurat  CltLength=12  MinVal=-0.05  MaxVal=0.05  MeanVal=0  VarVal=0.00025  RepMode=Not repeatable  rawSeed=1  IsInherit=off  SampMode=Discrete  SampTime=.001  SampFrame=1  DataType=Double  OutComplex=Real  OutputFrames=off
  Random Source{6..7,16..17} (4 alike) : dspsrcs4/Random Source  SrcType=Uniform  NormMethod=Ziggurat  CltLength=12  MinVal=-0.05  MaxVal=0.05  MeanVal=0  VarVal=1  RepMode=Not repeatable  rawSeed=1  IsInherit=off  SampMode=Discrete  SampTime=.001  SampFrame=1  DataType=Double  OutComplex=Real  OutputFrames=off
  Random Source18 : dspsrcs4/Random Source  Commented=on  SrcType=Gaussian  NormMethod=Ziggurat  CltLength=12  MinVal=-0.05  MaxVal=0.05  MeanVal=0  VarVal=0.00005  RepMode=Not repeatable  rawSeed=1  IsInherit=off  SampMode=Discrete  SampTime=.001  SampFrame=1  DataType=Double  OutComplex=Real  OutputFrames=off
  Random Source8 : dspsrcs4/Random Source  SrcType=Gaussian  NormMethod=Ziggurat  CltLength=12  MinVal=-0.01  MaxVal=0.01  MeanVal=0  VarVal=0.00005  RepMode=Not repeatable  rawSeed=1  IsInherit=off  SampMode=Discrete  SampTime=.001  SampFrame=1  DataType=Double  OutComplex=Real  OutputFrames=off
  Random Source9 : dspsrcs4/Random Source  SrcType=Gaussian  NormMethod=Ziggurat  CltLength=12  MinVal=-0.05  MaxVal=0.05  MeanVal=0  VarVal=0.00005  RepMode=Not repeatable  rawSeed=1  IsInherit=off  SampMode=Discrete  SampTime=.001  SampFrame=1  DataType=Double  OutComplex=Real  OutputFrames=off
  Resistor : ee_lib/Passive/Resistor  Commented=on  R=R Ohm  R_tol=5  enable_R_tol=0  tol_distribution=1  nSigma=4  enable_operating_limits=0  operating_limit_action=2  max_working_voltage=100 V  power_rating=1 W  enable_faults=0  fault_action=1  R_faulted=inf Ohm  enable_temporal_fault=0  t_fault=1 s  enable_behavioral_fault=0  max_permissible_current=1 A  t_fail_on_current=1 s  noise_mode=0  sample_time=1e-3 s  repeatability=1  auto_seed=3519391732  user_seed=0  Tdevice=25 degC  alpha=3.93e-3 1/K  Tmeas=25 degC  thermal_mass=100 J/K  power_derating_T1=70 degC  power_derating_T2=155 degC  operating_temperature_range_vec=[-50, 150] degC  temperature_specify=off  temperature_priority=High  temperature=298.15 K  temperature_nominal_specify=off  temperature_nominal_unit=K  temperature_nominal_value=1
  Resistor1 : ee_lib/Passive/Resistor  Commented=on  R=R Ohm  R_tol=5  enable_R_tol=0  tol_distribution=1  nSigma=4  enable_operating_limits=0  operating_limit_action=2  max_working_voltage=100 V  power_rating=1 W  enable_faults=0  fault_action=1  R_faulted=inf Ohm  enable_temporal_fault=0  t_fault=1 s  enable_behavioral_fault=0  max_permissible_current=1 A  t_fail_on_current=1 s  noise_mode=0  sample_time=1e-3 s  repeatability=1  auto_seed=2287600524  user_seed=0  Tdevice=25 degC  alpha=3.93e-3 1/K  Tmeas=25 degC  thermal_mass=100 J/K  power_derating_T1=70 degC  power_derating_T2=155 degC  operating_temperature_range_vec=[-50, 150] degC  temperature_specify=off  temperature_priority=High  temperature=298.15 K  temperature_nominal_specify=off  temperature_nominal_unit=K  temperature_nominal_value=1
  Resistor2 : ee_lib/Passive/Resistor  Commented=on  R=R Ohm  R_tol=5  enable_R_tol=0  tol_distribution=1  nSigma=4  enable_operating_limits=0  operating_limit_action=2  max_working_voltage=100 V  power_rating=1 W  enable_faults=0  fault_action=1  R_faulted=inf Ohm  enable_temporal_fault=0  t_fault=1 s  enable_behavioral_fault=0  max_permissible_current=1 A  t_fail_on_current=1 s  noise_mode=0  sample_time=1e-3 s  repeatability=1  auto_seed=355764756  user_seed=0  Tdevice=25 degC  alpha=3.93e-3 1/K  Tmeas=25 degC  thermal_mass=100 J/K  power_derating_T1=70 degC  power_derating_T2=155 degC  operating_temperature_range_vec=[-50, 150] degC  temperature_specify=off  temperature_priority=High  temperature=298.15 K  temperature_nominal_specify=off  temperature_nominal_unit=K  temperature_nominal_value=1
  Resistor3 : ee_lib/Passive/Resistor  R=R Ohm  R_tol=5  enable_R_tol=0  tol_distribution=1  nSigma=4  enable_operating_limits=0  operating_limit_action=2  max_working_voltage=100 V  power_rating=1 W  enable_faults=0  fault_action=1  R_faulted=inf Ohm  enable_temporal_fault=0  t_fault=1 s  enable_behavioral_fault=0  max_permissible_current=1 A  t_fail_on_current=1 s  noise_mode=0  sample_time=1e-3 s  repeatability=1  auto_seed=137400367  user_seed=0  Tdevice=25 degC  alpha=3.93e-3 1/K  Tmeas=25 degC  thermal_mass=100 J/K  power_derating_T1=70 degC  power_derating_T2=155 degC  operating_temperature_range_vec=[-50, 150] degC  temperature_specify=off  temperature_priority=High  temperature=298.15 K  temperature_nominal_specify=off  temperature_nominal_unit=K  temperature_nominal_value=1
  Resistor4 : ee_lib/Passive/Resistor  R=R Ohm  R_tol=5  enable_R_tol=0  tol_distribution=1  nSigma=4  enable_operating_limits=0  operating_limit_action=2  max_working_voltage=100 V  power_rating=1 W  enable_faults=0  fault_action=1  R_faulted=inf Ohm  enable_temporal_fault=0  t_fault=1 s  enable_behavioral_fault=0  max_permissible_current=1 A  t_fail_on_current=1 s  noise_mode=0  sample_time=1e-3 s  repeatability=1  auto_seed=2640174031  user_seed=0  Tdevice=25 degC  alpha=3.93e-3 1/K  Tmeas=25 degC  thermal_mass=100 J/K  power_derating_T1=70 degC  power_derating_T2=155 degC  operating_temperature_range_vec=[-50, 150] degC  temperature_specify=off  temperature_priority=High  temperature=298.15 K  temperature_nominal_specify=off  temperature_nominal_unit=K  temperature_nominal_value=1
  Resistor5 : ee_lib/Passive/Resistor  Commented=on  R=.5 Ohm  R_tol=5  enable_R_tol=0  tol_distribution=1  nSigma=4  enable_operating_limits=0  operating_limit_action=2  max_working_voltage=100 V  power_rating=1 W  enable_faults=0  fault_action=1  R_faulted=inf Ohm  enable_temporal_fault=0  t_fault=1 s  enable_behavioral_fault=0  max_permissible_current=1 A  t_fail_on_current=1 s  noise_mode=0  sample_time=1e-3 s  repeatability=1  auto_seed=1030432034  user_seed=0  Tdevice=25 degC  alpha=3.93e-3 1/K  Tmeas=25 degC  thermal_mass=100 J/K  power_derating_T1=70 degC  power_derating_T2=155 degC  operating_temperature_range_vec=[-50, 150] degC  temperature_specify=off  temperature_priority=High  temperature=298.15 K  temperature_nominal_specify=off  temperature_nominal_unit=K  temperature_nominal_value=1
  Resistor6 : ee_lib/Passive/Resistor  Commented=on  R=R Ohm  R_tol=5  enable_R_tol=0  tol_distribution=1  nSigma=4  enable_operating_limits=0  operating_limit_action=2  max_working_voltage=100 V  power_rating=1 W  enable_faults=0  fault_action=1  R_faulted=inf Ohm  enable_temporal_fault=0  t_fault=1 s  enable_behavioral_fault=0  max_permissible_current=1 A  t_fail_on_current=1 s  noise_mode=0  sample_time=1e-3 s  repeatability=1  auto_seed=529650792  user_seed=0  Tdevice=25 degC  alpha=3.93e-3 1/K  Tmeas=25 degC  thermal_mass=100 J/K  power_derating_T1=70 degC  power_derating_T2=155 degC  operating_temperature_range_vec=[-50, 150] degC  temperature_specify=off  temperature_priority=High  temperature=298.15 K  temperature_nominal_specify=off  temperature_nominal_unit=K  temperature_nominal_value=1
  Resistor7 : ee_lib/Passive/Resistor  Commented=on  R=R Ohm  R_tol=5  enable_R_tol=0  tol_distribution=1  nSigma=4  enable_operating_limits=0  operating_limit_action=2  max_working_voltage=100 V  power_rating=1 W  enable_faults=0  fault_action=1  R_faulted=inf Ohm  enable_temporal_fault=0  t_fault=1 s  enable_behavioral_fault=0  max_permissible_current=1 A  t_fail_on_current=1 s  noise_mode=0  sample_time=1e-3 s  repeatability=1  auto_seed=1038056169  user_seed=0  Tdevice=25 degC  alpha=3.93e-3 1/K  Tmeas=25 degC  thermal_mass=100 J/K  power_derating_T1=70 degC  power_derating_T2=155 degC  operating_temperature_range_vec=[-50, 150] degC  temperature_specify=off  temperature_priority=High  temperature=298.15 K  temperature_nominal_specify=off  temperature_nominal_unit=K  temperature_nominal_value=1
  Resistor8 : ee_lib/Passive/Resistor  Commented=on  R=R Ohm  R_tol=5  enable_R_tol=0  tol_distribution=1  nSigma=4  enable_operating_limits=0  operating_limit_action=2  max_working_voltage=100 V  power_rating=1 W  enable_faults=0  fault_action=1  R_faulted=inf Ohm  enable_temporal_fault=0  t_fault=1 s  enable_behavioral_fault=0  max_permissible_current=1 A  t_fail_on_current=1 s  noise_mode=0  sample_time=1e-3 s  repeatability=1  auto_seed=1734789456  user_seed=0  Tdevice=25 degC  alpha=3.93e-3 1/K  Tmeas=25 degC  thermal_mass=100 J/K  power_derating_T1=70 degC  power_derating_T2=155 degC  operating_temperature_range_vec=[-50, 150] degC  temperature_specify=off  temperature_priority=High  temperature=298.15 K  temperature_nominal_specify=off  temperature_nominal_unit=K  temperature_nominal_value=1
  Rotational Electromechanical Converter : fl_lib/Electrical/Electrical Elements/Rotational Electromechanical Converter  Commented=on  K=0.1 V/(rad/s)  i_specify=off  i_priority=None  i=0 A  i_nominal_specify=off  i_nominal_unit=A  i_nominal_value=1  v_specify=off  v_priority=None  v=0 V  v_nominal_specify=off  v_nominal_unit=V  v_nominal_value=1  t_specify=off  t_priority=None  t=0 N*m  t_nominal_specify=off  t_nominal_unit=N*m  t_nominal_value=1  w_specify=off  w_priority=None  w=0 rad/s  w_nominal_specify=off  w_nominal_unit=rad/s  w_nominal_value=1
  Rotational Damper : fl_lib/Mechanical/Rotational Elements/Rotational Damper  Commented=on  D=b N*m/(rad/s)  w_specify=off  w_priority=None  w=0 rad/s  w_nominal_specify=off  w_nominal_unit=rad/s  w_nominal_value=1  t_specify=off  t_priority=None  t=0 N*m  t_nominal_specify=off  t_nominal_unit=N*m  t_nominal_value=1
  Rotational Damper1 : fl_lib/Mechanical/Rotational Elements/Rotational Damper  Commented=on  D=b N*m/(rad/s)  w_specify=off  w_priority=None  w=0 rad/s  w_nominal_specify=off  w_nominal_unit=rad/s  w_nominal_value=1  t_specify=off  t_priority=None  t=0 N*m  t_nominal_specify=off  t_nominal_unit=N*m  t_nominal_value=1
  Scope{1..9,17,21..25,38..44,47..61,70} (38 alike) : Scope  Commented=on  NumInputPorts=2
  Scope{10..16,18..20,26..30,32..37} (21 alike) : Scope  Commented=on  NumInputPorts=3
  Scope31 : Scope  Commented=on  NumInputPorts=4
  Scope45 : Scope
  Scope{46,62..69} (9 alike) : Scope  NumInputPorts=2
  Simulink-PS Converter : nesl_utility/Simulink-PS Converter  Commented=on  PhysicalDomain=network_engine_domain  SubClassName=ps_input  LeftPortType=input  RightPortType=output  PseudoPeriodic=off  Frequencies=[]  NoiseDistribution=none  NoiseParameters=[]  Unit=N*m  AffineConversion=off  FilteringAndDerivatives=provide  SimscapeFilterOrder=1  InputFilterTimeConstant=0.001  UdotUserProvided=0
  Simulink-PS Converter{1..4} (4 alike) : nesl_utility/Simulink-PS Converter  Commented=on  PhysicalDomain=network_engine_domain  SubClassName=ps_input  LeftPortType=input  RightPortType=output  PseudoPeriodic=off  Frequencies=[]  NoiseDistribution=none  NoiseParameters=[]  Unit=1  AffineConversion=off  FilteringAndDerivatives=provide  SimscapeFilterOrder=1  InputFilterTimeConstant=0.001  UdotUserProvided=0
  Simulink-PS Converter5 : nesl_utility/Simulink-PS Converter  Commented=on  PhysicalDomain=network_engine_domain  SubClassName=ps_input  LeftPortType=input  RightPortType=output  PseudoPeriodic=off  Frequencies=[]  NoiseDistribution=none  NoiseParameters=[]  Unit=N*m  AffineConversion=off  FilteringAndDerivatives=provide  SimscapeFilterOrder=1  InputFilterTimeConstant=0.001  UdotUserProvided=0
  Sin{1..9,11..12} (11 alike) : Trigonometry  Commented=on
  Sin10 : Trigonometry
  Sine Wave{,2,8,10} (4 alike) : Sin  Commented=on  Amplitude=20  Frequency=2*pi*310  SampleTime=0
  Sine Wave{1,3,9,11} (4 alike) : Sin  Commented=on  Amplitude=20  Frequency=2*pi*310  Phase=-pi/2  SampleTime=0
  Sine Wave12 : Sin  Commented=on  Amplitude=20  Bias=24  Frequency=2*pi*50  SampleTime=0
  Sine Wave13 : Sin  Commented=on  Amplitude=20  Bias=24  Frequency=2*pi*50  Phase=-pi/2  SampleTime=0
  Sine Wave4 : Sin  Commented=on  Amplitude=24  Frequency=2*pi*50  SampleTime=0
  Sine Wave5 : Sin  Commented=on  Amplitude=24  Frequency=2*pi*50  Phase=-pi/2  SampleTime=0
  Sine Wave6 : Sin  Commented=on  Amplitude=5  Frequency=2*pi*50  SampleTime=0
  Sine Wave7 : Sin  Commented=on  Amplitude=5  Frequency=2*pi*50  Phase=-pi/2  SampleTime=0
  Solver Configuration{,1..4} (5 alike) : nesl_utility/Solver Configuration  Commented=on  PhysicalDomain=network_engine_domain  SubClassName=solver  LeftPortType=input  RightPortType=generic  Tones=[]  Harmonics=[]  SimulateNoise=off  Profile=off  UseLocalSampling=off  EnableSwitchedLinearOptims=on  FrequencyDomain=off  UseCCode=off  RelTol=0.001  AbsTol=1e-06  MinStep=1e-09  ToWorkspace=off  RevertToSquareIcSolve=off  NumHomotopyIterations=100  PhasorMode=off  PhasorModeNumHarmonics=1  DoDC=off  ResidualTolerance=1e-09  UseLocalSolver=off  LocalSolverChoice=NE_BACKWARD_EULER_ADVANCER  LocalSolverSampleTime=0.001  DoFixedCost=off  MaxNonlinIter=3  MaxModeIter=2  ComputeImpulses=off  ImpulseIterations=2  LinearAlgebra=auto  EquationFormulation=NE_TIME_EF  DelaysMemoryBudget=1024  AutomaticFiltering=on  FilteringTimeConstant=0.001  PartitionStorageMethod=AS_NEEDED  PartitionMemoryBudget=1024  PartitionMethod=ROBUST
  Step1 : Step  Commented=on  Time=0.01  After=U  SampleTime=0
  Step10 : Step  Commented=on  Time=0.5  After=3  SampleTime=0
  Step{6,9,11,16,18} (5 alike) : Step  Commented=on  Time=7  After=T_load  SampleTime=0
  Step12 : Step  Commented=on  Time=0.5  After=3  SampleTime=0
  Step13 : Step  Time=0.5  After=3  SampleTime=0
  Step14 : Step  Time=0.75  After=T_load*10  SampleTime=0
  Step15 : Step  Commented=on  Time=0.5  After=3  SampleTime=0
  Step17 : Step  Commented=on  Time=0.5  SampleTime=0
  Step2 : Step  Commented=on  Time=5  After=-T_load  SampleTime=0
  Step3 : Step  Commented=on  Time=4  After=T_load  SampleTime=0
  Step4 : Step  Commented=on  Time=5  After=-T_load  SampleTime=0
  Step5 : Step  Commented=on  Time=4  After=T_load  SampleTime=0
  Step7 : Step  After=4  SampleTime=0
  Step8 : Step  Commented=on  After=3  SampleTime=0
  Stepper Motor : powerlib/Machines/Stepper Motor  Commented=on  MotorType=Permanent-magnet / Hybrid  NumberOfPhases_1=2  NumberOfPhases_2=3  PresetModel_1=<empty>  PresetModel_2=<empty>  L=10e-3  Lmax=10e-3  Lmin=2e-3  R=1.2  Step_angle=30  Psim=0.04  Tdm=0.02  J=1e-4/5  B=1e-3  w0=0  pos0=0  TsPowergui=0  TsBlock=-1
      settings: SourceProductBaseCode=PS
  Stepper Motor1 : ee_lib/Electromechanical/Reluctance & Stepper/Stepper Motor  Commented=on  step_or_av=1  w_vec=[0, 1000, 3000] rpm  T_vec=[2, 2, 1] N*m  assert_if_slipping=0  J_total=1e-4 kg*m^2  max_step_rate=10 Hz  Ra=0.55 Ohm  La=1.5e-3 H  Km=0.19 N*m/A  Td=0 N*m  Rm=inf Ohm  Step=1.8 deg  J=4.5e-5 kg*m^2  B=8.0e-4 N*m/(rad/s)  speed0=0 rpm  theta0=0 deg  alpha=[.00393, .00393] 1/K  Tmeas=25 degC  T_vec2=[1.7, 1.7, .85] N*m  Tmeas2=125 degC  half_stepping=0  thermal_masses=[100, 100] J/K  initial_temperatures=[25, 25] degC  rotor_thermal_mass=50 J/K  rotor_initial_temperature=25 degC  Rm_percent_rotor=90
      settings: SourceProductBaseCode=PS  InternalSimscapePortConfiguration="{\"Bottom\":[],\"Left\":[{\"id\":\"pA\",\"label\":\"A+\",\"type\":\"foundation.electrical.electrical\"},{\"id\":\"nA\",\"label\":\"A-\",\"type\":\"foundation.electrical.electrical\"},{\"id\":\"pB\",\"label\":\"B+\",\"type\":\"foundation.electrical.electrical\"},{\"id\":\"nB\",\"label\":\"B-\",\"type\":\"foundation.electrical.electrical\"}],\"Right\":[{\"id\":\"R\",\"label\":\"R\",\"type\":\"foundation.mechanical.rotational.rotational\"},{\"id\":\"C\",\"label\":\"C\",\"type\":\"foundation.mechanical.rotational.rotational\"}],\"Top\":[]}"
  Subsystem : Subsystem
  Sum{,1,80..82} (5 alike) : Sum  Inputs=|++
  Sum{6..13,17..20,22,24..25,27..28,30,32,36..37,39..40,42,46..48,53,57,59,63..64,66,70..73,85,89,92,94,98} (42 alike) : Sum  Commented=on  Inputs=|+-
  Sum{2..5,15..16,23,34..35,38,43..45,54..56,60..62,67..69,74..76,86..88,90..91,95..97,99..100} (35 alike) : Sum  Commented=on  Inputs=|++
  Sum{14,33,41,58,65,84,93} (7 alike) : Sum  Commented=on  Inputs=-+-
  Sum21 : Sum  Commented=on  Inputs=|-+
  Sum26 : Sum  Commented=on  Inputs=|-+
  Sum29 : Sum  Commented=on  Inputs=-+|
  Sum31 : Sum  Commented=on  Inputs=-+|
  Sum{49..52,77,79,83} (7 alike) : Sum  Inputs=|+-
  Sum78 : Sum  Inputs=-+-
  Synchronous Reluctance Machine : ee_lib/Electromechanical/Reluctance & Stepper/Synchronous Reluctance Machine  Commented=on  nPolePairs=4  stator_param=ee.enum.statorparam.LdLqL0  machine_param=ee.enum.dqparameterization.constant  Ld=0.0031 H  Lq=0.004 H  idVec=[-200, 0, 200] A  iqVec=[-200, 0, 200] A  LdMatrix=0.0031 * ones(3, 3) H  LqMatrix=0.004 * ones(3, 3) H  L0=0.0005 H  Ls=0.0025 H  Lm=-0.0003 H  Ms=0.0010 H  Rs=0.7 Ohm  zero_sequence=ee.enum.park.zerosequence.include  J=0.01 kg*m^2  lam=0 N*m/(rad/s)  axes_param=ee.enum.rotorangle.daxis  i_d_specify=off  i_d_priority=None  i_d=0 A  i_d_nominal_specify=off  i_d_nominal_unit=A  i_d_nominal_value=1  i_q_specify=off  i_q_priority=None  i_q=0 A  i_q_nominal_specify=off  i_q_nominal_unit=A  i_q_nominal_value=1  torque_specify=off  torque_priority=None  torque=0 N*m  torque_nominal_specify=off  torque_nominal_unit=N*m  torque_nominal_value=1  angular_velocity_specify=off  angular_velocity_priority=High  angular_velocity=0 rpm  angular_velocity_nominal_specify=off  angular_velocity_nominal_unit=rpm  angular_velocity_nominal_value=1  angular_position_specify=off  angular_position_priority=High  angular_position=0 deg  angular_position_nominal_specify=off  angular_position_nominal_unit=deg  angular_position_nominal_value=1
      settings: SourceProductBaseCode=PS  InternalSimscapePortConfiguration="{\"Bottom\":[],\"Left\":[{\"id\":\"N\",\"label\":\"~\",\"type\":\"foundation.electrical.three_phase\"},{\"id\":\"n\",\"label\":\"n\",\"type\":\"foundation.electrical.electrical\"}],\"Right\":[{\"id\":\"R\",\"label\":\"R\",\"type\":\"foundation.mechanical.rotational.rotational\"},{\"id\":\"C\",\"label\":\"C\",\"type\":\"foundation.mechanical.rotational.rotational\"}],\"Top\":[]}"
  Terminator : Terminator  Commented=on
  Terminator1 : Terminator  Commented=on
  To Workspace : ToWorkspace  VariableName=simout  SaveFormat=Timeseries  SampleTime=-1
  To Workspace1 : ToWorkspace  VariableName=simout1  SaveFormat=Timeseries  SampleTime=-1
  To Workspace2 : ToWorkspace  Commented=on  VariableName=simout2  SaveFormat=Timeseries  SampleTime=-1
  To Workspace3 : ToWorkspace  Commented=on  VariableName=simout3  SaveFormat=Timeseries  SampleTime=-1
  To Workspace4 : ToWorkspace  Commented=on  VariableName=simout4  SaveFormat=Timeseries  SampleTime=-1
  To Workspace5 : ToWorkspace  Commented=on  VariableName=simout5  SaveFormat=Timeseries  SampleTime=-1
  To Workspace6 : ToWorkspace  Commented=on  VariableName=simout6  SaveFormat=Timeseries  SampleTime=-1
  Two-phase SVM : MATLAB Function  Commented=on  TreatAsAtomicUnit=on
  Two-phase SVM1 : MATLAB Function  Commented=on  TreatAsAtomicUnit=on
  Two-phase SVM2 : MATLAB Function  Commented=on  TreatAsAtomicUnit=on
  Two-phase SVM3 : MATLAB Function  Commented=on  TreatAsAtomicUnit=on
  Two-phase SVM4 : MATLAB Function  Commented=on  TreatAsAtomicUnit=on
  Voltage Measurement : powerlib/Measurements/Voltage Measurement  Commented=on  PhasorSimulation=off  OutputType=Complex  PSBequivalent=0
  Voltage Sensor{,1..9} (10 alike) : fl_lib/Electrical/Electrical Sensors/Voltage Sensor  Commented=on
  Voltage Source : ee_lib/Sources/Voltage Source  Commented=on  dc_voltage=0 V  ac_voltage=24 V  ac_shift=0 rad  ac_frequency=310 Hz  noise_mode=0  PSD=0 V^2/Hz  repeatability=1  auto_seed=292176722  user_seed=0  sample_time=1e-3 s  i_specify=off  i_priority=None  i=0 A  i_nominal_specify=off  i_nominal_unit=A  i_nominal_value=1  v_specify=off  v_priority=None  v=0 V  v_nominal_specify=off  v_nominal_unit=V  v_nominal_value=1
  Voltage Source1 : ee_lib/Sources/Voltage Source  Commented=on  dc_voltage=0 V  ac_voltage=24 V  ac_shift=-90 deg  ac_frequency=310 Hz  noise_mode=0  PSD=0 V^2/Hz  repeatability=1  auto_seed=2902803550  user_seed=0  sample_time=1e-3 s  i_specify=off  i_priority=None  i=0 A  i_nominal_specify=off  i_nominal_unit=A  i_nominal_value=1  v_specify=off  v_priority=None  v=0 V  v_nominal_specify=off  v_nominal_unit=V  v_nominal_value=1
  Voltage Source2 : ee_lib/Sources/Voltage Source  Commented=on  dc_voltage=0 V  ac_voltage=24 V  ac_shift=0 rad  ac_frequency=310 Hz  noise_mode=0  PSD=0 V^2/Hz  repeatability=1  auto_seed=2857547874  user_seed=0  sample_time=1e-3 s  i_specify=off  i_priority=None  i=0 A  i_nominal_specify=off  i_nominal_unit=A  i_nominal_value=1  v_specify=off  v_priority=None  v=0 V  v_nominal_specify=off  v_nominal_unit=V  v_nominal_value=1
  Voltage Source3 : ee_lib/Sources/Voltage Source  Commented=on  dc_voltage=24 V  ac_voltage=0 V  ac_shift=0 rad  ac_frequency=60 Hz  noise_mode=0  PSD=0 V^2/Hz  repeatability=1  auto_seed=1284946224  user_seed=0  sample_time=1e-3 s  i_specify=off  i_priority=None  i=0 A  i_nominal_specify=off  i_nominal_unit=A  i_nominal_value=1  v_specify=off  v_priority=None  v=0 V  v_nominal_specify=off  v_nominal_unit=V  v_nominal_value=1
  Voltage Source4 : ee_lib/Sources/Voltage Source  Commented=on  dc_voltage=0 V  ac_voltage=3 V  ac_shift=0 rad  ac_frequency=310 Hz  noise_mode=0  PSD=0 V^2/Hz  repeatability=1  auto_seed=1442963394  user_seed=0  sample_time=1e-3 s  i_specify=off  i_priority=None  i=0 A  i_nominal_specify=off  i_nominal_unit=A  i_nominal_value=1  v_specify=off  v_priority=None  v=0 V  v_nominal_specify=off  v_nominal_unit=V  v_nominal_value=1
  Voltage Source5 : ee_lib/Sources/Voltage Source  Commented=on  dc_voltage=24 V  ac_voltage=0 V  ac_shift=0 rad  ac_frequency=60 Hz  noise_mode=0  PSD=0 V^2/Hz  repeatability=1  auto_seed=3367373959  user_seed=0  sample_time=1e-3 s  i_specify=off  i_priority=None  i=0 A  i_nominal_specify=off  i_nominal_unit=A  i_nominal_value=1  v_specify=off  v_priority=None  v=0 V  v_nominal_specify=off  v_nominal_unit=V  v_nominal_value=1
  Voltage Source6 : ee_lib/Sources/Voltage Source  Commented=on  dc_voltage=24 V  ac_voltage=0 V  ac_shift=0 rad  ac_frequency=60 Hz  noise_mode=0  PSD=0 V^2/Hz  repeatability=1  auto_seed=1725752364  user_seed=0  sample_time=1e-3 s  i_specify=off  i_priority=None  i=0 A  i_nominal_specify=off  i_nominal_unit=A  i_nominal_value=1  v_specify=off  v_priority=None  v=0 V  v_nominal_specify=off  v_nominal_unit=V  v_nominal_value=1
  Voltage Source7 : ee_lib/Sources/Voltage Source  Commented=on  dc_voltage=0 V  ac_voltage=24 V  ac_shift=0 rad  ac_frequency=310 Hz  noise_mode=0  PSD=0 V^2/Hz  repeatability=1  auto_seed=414269032  user_seed=0  sample_time=1e-3 s  i_specify=off  i_priority=None  i=0 A  i_nominal_specify=off  i_nominal_unit=A  i_nominal_value=1  v_specify=off  v_priority=None  v=0 V  v_nominal_specify=off  v_nominal_unit=V  v_nominal_value=1
  Voltage Source8 : ee_lib/Sources/Voltage Source  Commented=on  dc_voltage=0 V  ac_voltage=24 V  ac_shift=-90 deg  ac_frequency=310 Hz  noise_mode=0  PSD=0 V^2/Hz  repeatability=1  auto_seed=566820976  user_seed=0  sample_time=1e-3 s  i_specify=off  i_priority=None  i=0 A  i_nominal_specify=off  i_nominal_unit=A  i_nominal_value=1  v_specify=off  v_priority=None  v=0 V  v_nominal_specify=off  v_nominal_unit=V  v_nominal_value=1
  Zero-Order Hold{,1,4..9} (8 alike) : ZeroOrderHold  Commented=on  SampleTime=25e-6
  Zero-Order Hold{10..11,22..29,36..39} (14 alike) : ZeroOrderHold  Commented=on  SampleTime=50e-6
  Zero-Order Hold{12..13,40..41} (4 alike) : ZeroOrderHold  Commented=on  SampleTime=5e-6
  Zero-Order Hold{14..19,42..47} (12 alike) : ZeroOrderHold  Commented=on  SampleTime=20e-6
  Zero-Order Hold2 : ZeroOrderHold  Commented=on  SampleTime=12.5e-6
  Zero-Order Hold{20..21,30..35} (8 alike) : ZeroOrderHold  SampleTime=50e-6
  Zero-Order Hold3 : ZeroOrderHold  Commented=on  SampleTime=12.5e-6
  wires:
  From1/1 -> MATLAB Function1/1(X_q), Scope1/1
  From/1 -> MATLAB Function1/2(X_d), Scope1/2
  MATLAB Function1/1(X_a) -> Scope2/1
  MATLAB Function1/2(X_b) -> Scope2/2
  From5/1 -> MATLAB Function1/3(theta_e), MATLAB Function2/3(theta_e)
  Step2/1 -> Scope6/2, Simulink-PS Converter/1
  PS-Simulink Converter/1 -> Scope3/1
  PS-Simulink Converter1/1 -> Scope3/2
  PS-Simulink Converter2/1 -> Goto4/1
  PS-Simulink Converter3/1 -> Goto5/1
  PS-Simulink Converter4/1 -> Scope4/1
  PS-Simulink Converter5/1 -> Scope4/2
  MATLAB Function2/1(X_a) -> Scope5/1
  MATLAB Function2/2(X_b) -> Scope5/2
  PS-Simulink Converter6/1 -> Scope6/1
  PS-Simulink Converter10/1 -> Scope8/1
  PS-Simulink Converter11/1 -> Scope8/2
  PS-Simulink Converter9/1 -> Scope7/2
  PS-Simulink Converter8/1 -> Scope7/1
  PS-Simulink Converter13/1 -> Scope9/1
  PS-Simulink Converter12/1 -> Scope9/2
  Two-phase SVM/1(DC_PWM1) -> PWM Generator1/1
  Two-phase SVM/2(DC_PWM3) -> PWM Generator2/1
  Two-phase SVM/3(DC_PWM5) -> PWM Generator3/1
  Two-phase SVM/4(DC_PWM7) -> PWM Generator4/1
  PWM Generator1/1 -> Sum7/1, Scope11/1, Simulink-PS Converter1/1
  PWM Generator2/1 -> Scope11/2, Sum7/2, Simulink-PS Converter2/1
  PWM Generator3/1 -> Sum8/1, Scope13/1, Simulink-PS Converter3/1
  PWM Generator4/1 -> Sum8/2, Scope13/2, Simulink-PS Converter4/1
  Constant/1 -> Two-phase SVM/3(U)
  Constant1/1 -> Two-phase SVM/4(Ts)
  Sine Wave/1 -> Two-phase SVM/1(Ua), Scope12/1, Scope10/1
  Sine Wave1/1 -> Scope12/2, Two-phase SVM/2(Ub)
  PS-Simulink Converter7/1 -> Scope10/2
  PS-Simulink Converter14/1 -> Scope10/3
  Sum7/1 -> Scope11/3
  Sum8/1 -> Scope13/3
  Sum10/1 -> Scope16/3
  Sum9/1 -> Scope14/3
  PWM Generator8/1 -> Sum11/2, Sum10/2, Scope16/2
  Constant3/1 -> Two-phase SVM1/4(Ts)
  PWM Generator5/1 -> Sum12/1, Sum9/1, Scope14/1
  MATLAB Function4/1(X_a) -> Two-phase SVM1/1(Ua), Scope15/1
  Two-phase SVM1/3(DC_PWM5) -> PWM Generator7/1
  MATLAB Function4/2(X_b) -> Scope15/2, Two-phase SVM1/2(Ub)
  Constant2/1 -> Two-phase SVM1/3(U)
  PWM Generator7/1 -> Sum11/1, Sum10/1, Scope16/1
  Two-phase SVM1/2(DC_PWM3) -> PWM Generator6/1
  Two-phase SVM1/1(DC_PWM1) -> PWM Generator5/1
  PWM Generator6/1 -> Scope14/2, Sum9/2, Sum12/2
  Two-phase SVM1/4(DC_PWM7) -> PWM Generator8/1
  Sum11/1 -> Gain15/1
  From7/1 -> MATLAB Function2/2(X_d)
  From6/1 -> MATLAB Function2/1(X_q)
  Gain12/1 -> MATLAB Function4/2(X_d)
  From8/1 -> MATLAB Function4/3(theta_e)
  Sum12/1 -> Gain14/1
  Gain14/1 -> MATLAB Function5/1(X_a)
  Gain15/1 -> MATLAB Function5/2(X_b)
  From9/1 -> MATLAB Function5/3(theta_e)
  Step1/1 -> MATLAB Function4/1(X_q)
  Gain17/1 -> Sum13/2
  Gain18/1 -> Goto9/1
  Integrator5/1 -> Scope17/1, Gain17/1, Goto8/1, Integrator4/1
  Integrator4/1 -> Scope17/2, Gain18/1, Gain20/1
  Sum13/1 -> Gain16/1
  Sin1/1 -> Gain19/1
  Sum14/1 -> Sum13/1
  Gain16/1 -> Integrator5/1
  Step3/1 -> Sum14/1
  Gain20/1 -> Sin1/1
  From10/1 -> Sin2/1
  Sin2/1 -> Product2/1
  Product2/1 -> Sum15/1
  Gain21/1 -> Product2/2
  Integrator7/1 -> Product3/2, Scope22/2, Gain30/1
  From11/1 -> Cos1/1
  Product3/1 -> Sum15/2
  Cos1/1 -> Product3/1
  Sum15/1 -> Gain22/1
  Integrator6/1 -> Scope22/1, Gain24/1, Gain21/1
  Gain23/1 -> Integrator6/1
  Sum16/1 -> Gain23/1
  Sum17/1 -> Sum16/2
  Gain24/1 -> Sum17/2
  From12/1 -> Gain25/1
  Sin4/1 -> Product4/1
  Product4/1 -> Sum17/1
  Gain25/1 -> Product4/2
  From13/1 -> Sin4/1
  PWM Generator11/1 -> Sum19/1, Scope20/1
  Sine Wave5/1 -> Zero-Order Hold1/1
  Two-phase SVM2/2(DC_PWM3) -> Sum18/2, Scope26/2, PWM Generator10/1
  Sum20/1 -> Gain26/1, Scope18/3
  PWM Generator10/1 -> Sum20/2, Scope18/2
  Two-phase SVM2/4(DC_PWM7) -> PWM Generator12/1
  PWM Generator12/1 -> Sum19/2, Scope20/2
  Constant5/1 -> Two-phase SVM2/4(Ts)
  Two-phase SVM2/1(DC_PWM1) -> Sum18/1, Scope26/1, PWM Generator9/1
  Sum19/1 -> Scope20/3, Gain27/1
  Constant4/1 -> Two-phase SVM2/3(U)
  Two-phase SVM2/3(DC_PWM5) -> PWM Generator11/1
  PWM Generator9/1 -> Sum20/1, Scope18/1
  Sine Wave4/1 -> Zero-Order Hold/1
  Product5/1 -> Sum23/1
  From15/1 -> Cos/1
  Cos/1 -> Product5/1
  Gain30/1 -> Sum23/2
  Gain29/1 -> Integrator7/1
  Gain31/1 -> Product5/2
  From14/1 -> Gain31/1
  Sum22/1 -> Gain29/1
  Sum23/1 -> Sum22/2
  PS-Simulink Converter15/1 -> Scope23/1
  PS-Simulink Converter17/1 -> Goto10/1
  PS-Simulink Converter21/1 -> Scope25/1
  PS-Simulink Converter19/1 -> Scope24/1
  PS-Simulink Converter16/1 -> Scope23/2
  PS-Simulink Converter18/1 -> Goto11/1
  Step4/1 -> Scope25/2, Simulink-PS Converter5/1
  PS-Simulink Converter20/1 -> Scope24/2
  Gain22/1 -> Sum14/2
  Gain19/1 -> Sum14/3
  Zero-Order Hold/1 -> Scope19/1, Scope31/1, Two-phase SVM2/1(Ua)
  Zero-Order Hold1/1 -> Scope19/2, Scope31/2, Two-phase SVM2/2(Ub)
  Sum18/1 -> Scope31/3, Scope26/3
  Constant7/1 -> Two-phase SVM3/4(Ts)
  Constant6/1 -> Two-phase SVM3/3(U)
  Sine Wave8/1 -> Zero-Order Hold2/1
  Sine Wave9/1 -> Zero-Order Hold3/1
  Zero-Order Hold3/1 -> Scope27/2, Two-phase SVM3/2(Ub)
  Zero-Order Hold2/1 -> Scope27/1, Two-phase SVM3/1(Ua)
  Sum21/1 -> Scope30/3
  PWM Generator16/1 -> Sum25/1, Scope28/1
  Two-phase SVM3/1(DC_PWM1) -> Sum21/1, Scope30/1, PWM Generator16/1
  PWM Generator15/1 -> Sum24/2, Scope29/2
  Sum24/1 -> Scope29/3, Gain32/1
  PWM Generator13/1 -> Sum25/2, Scope28/2
  Two-phase SVM3/3(DC_PWM5) -> PWM Generator14/1
  Sum25/1 -> Gain28/1, Scope28/3
  Two-phase SVM3/2(DC_PWM3) -> Sum21/2, Scope30/2, PWM Generator13/1
  PWM Generator14/1 -> Sum24/1, Scope29/1
  Two-phase SVM3/4(DC_PWM7) -> PWM Generator15/1
  Sine Wave7/1 -> Zero-Order Hold5/1
  Sine Wave6/1 -> Zero-Order Hold4/1
  Zero-Order Hold4/1 -> Scope21/1, Sum16/1
  Zero-Order Hold5/1 -> Scope21/2, Sum22/1
  Gain26/1 -> Terminator/1
  Gain27/1 -> Terminator1/1
  PWM Generator18/1 -> Sum27/1, Scope34/1
  Two-phase SVM4/2(DC_PWM3) -> Sum26/2, Scope35/2, PWM Generator17/1
  Two-phase SVM4/3(DC_PWM5) -> PWM Generator18/1
  PWM Generator19/1 -> Sum27/2, Scope34/2
  PWM Generator17/1 -> Sum28/2, Scope33/2
  Sum27/1 -> Scope34/3, Gain34/1
  Zero-Order Hold6/1 -> Scope32/1, Two-phase SVM4/1(Ua)
  Sum28/1 -> Gain33/1, Scope33/3
  Two-phase SVM4/1(DC_PWM1) -> Sum26/1, Scope35/1, PWM Generator20/1
  Two-phase SVM4/4(DC_PWM7) -> PWM Generator19/1
  PWM Generator20/1 -> Sum28/1, Scope33/1
  Sine Wave11/1 -> Zero-Order Hold7/1
  Zero-Order Hold7/1 -> Scope32/2, Two-phase SVM4/2(Ub)
  Constant10/1 -> Two-phase SVM4/3(U)
  Constant11/1 -> Two-phase SVM4/4(Ts)
  Sum26/1 -> Scope35/3
  Sine Wave10/1 -> Zero-Order Hold6/1
  Sine Wave12/1 -> Scope37/1, Zero-Order Hold8/1
  Sine Wave13/1 -> Zero-Order Hold9/1
  Zero-Order Hold8/1 -> Divide/1
  Zero-Order Hold9/1 -> Divide1/1
  Constant15/1 -> Divide1/2, Divide/2
  Divide/1 -> PWM Generator21/1, Sum29/1, Scope36/3
  Constant14/1 -> Sum29/2
  Sum31/1 -> PWM Generator24/1
  Constant16/1 -> Sum31/2
  Divide1/1 -> PWM Generator23/1, Sum31/1
  Sum30/1 -> Gain48/1
  Sum35/1 -> Gain42/1
  From17/1 -> Cos3/1
  Integrator9/1 -> Scope38/1, Gain36/1, Goto12/1, Integrator8/1
  Sum37/1 -> Gain45/1
  Sum34/1 -> Gain41/1
  Gain41/1 -> Sum33/2
  From18/1 -> Gain44/1
  Sin3/1 -> Gain38/1
  Product8/1 -> Sum36/1
  Step5/1 -> Sum33/1
  Cos3/1 -> Product7/1
  Product6/1 -> Sum34/1
  Gain37/1 -> Goto13/1
  Gain47/1 -> Product9/2
  Gain36/1 -> Sum32/2
  Sum38/1 -> Sum37/2
  Cos2/1 -> Product9/1
  Sum39/1 -> Gain49/1
  Product9/1 -> Sum38/1
  From21/1 -> Cos2/1
  Gain45/1 -> Integrator11/1
  Integrator11/1 -> Product7/2, Scope40/2, Gain46/1
  From19/1 -> Sin6/1
  Gain43/1 -> Sum36/2
  Gain38/1 -> Sum33/3
  Gain35/1 -> Integrator9/1
  Sum36/1 -> Sum35/2
  Integrator10/1 -> Scope40/1, Gain43/1, Gain40/1
  From20/1 -> Gain47/1
  Sin6/1 -> Product8/1
  Gain40/1 -> Product6/2
  Sin5/1 -> Product6/1
  From16/1 -> Sin5/1
  Gain42/1 -> Integrator10/1
  Sum32/1 -> Gain35/1
  Sum33/1 -> Sum32/1
  Gain46/1 -> Sum38/2
  Product7/1 -> Sum34/2
  Integrator8/1 -> Scope38/2, Gain37/1, Gain39/1
  Gain39/1 -> Sin3/1
  Gain44/1 -> Product8/2
  PWM Generator21/1 -> Scope36/1, Sum30/1
  PWM Generator24/1 -> Sum39/2
  PWM Generator23/1 -> Sum39/1
  Gain48/1 -> Sum35/1, Scope37/2, Scope39/1
  Gain49/1 -> Sum37/1, Scope39/2
  PWM Generator22/1 -> Sum30/2, Scope36/2
  Sum29/1 -> PWM Generator22/1
  From27/1 -> MATLAB Function9/3(theta_e), MATLAB Function10/3(theta_e)
  Sum46/1 -> Sum44/2
  Sum43/1 -> Sum42/2
  Gain50/1 -> Integrator13/1
  From26/1 -> Product11/2
  From29/1 -> Scope47/2, MATLAB Function10/2(X_d)
  From22/1 -> MATLAB Function9/2(X_d), Scope42/2
  Integrator12/1 -> Scope41/2, Gain54/1, Gain56/1
  Sum47/1 -> Zero-Order Hold11/1, Goto19/1
  From28/1 -> MATLAB Function10/1(X_q), Scope47/1
  Gain55/1 -> Sum41/3
  MATLAB Function9/2(X_b) -> Scope43/2
  MATLAB Function10/1(X_a) -> Scope44/1
  Integrator13/1 -> Scope41/1, Gain51/1, Goto16/1, Integrator12/1
  Integrator15/1 -> Gain52/1, Zero-Order Hold23/1, Product10/2, Goto14/1
  MATLAB Function10/2(X_b) -> Scope44/2
  From23/1 -> MATLAB Function9/1(X_q), Scope42/1
  MATLAB Function9/1(X_a) -> Scope43/1
  From25/1 -> Product11/1
  Gain52/1 -> Sum46/2
  Sum41/1 -> Sum40/1
  Product11/1 -> Gain53/1
  From24/1 -> Product10/1, Gain62/1
  Gain59/1 -> Sum43/2
  Sum44/1 -> Gain60/1
  Gain53/1 -> Sum55/2, Sum46/1
  Gain60/1 -> Integrator15/1
  Gain62/1 -> Sum45/1
  Gain61/1 -> Sum45/2
  Sum45/1 -> Sum56/2, Sum43/1
  Gain54/1 -> Goto17/1
  Gain57/1 -> Sum41/2
  Product10/1 -> Gain61/1
  Sum40/1 -> Gain50/1
  Step6/1 -> Sum41/1
  Sum42/1 -> Gain58/1
  Integrator14/1 -> Gain57/1, Gain59/1, Goto15/1
  Gain56/1 -> Sin7/1
  Gain51/1 -> Sum40/2
  Gain58/1 -> Integrator14/1
  Sin7/1 -> Gain55/1
  PID Controller4/1 -> Sum47/1
  Sum48/1 -> PID Controller4/1
  Constant17/1 -> Sum48/1
  Sum49/1 -> Gain64/1
  Gain64/1 -> Integrator16/1
  Integrator16/1 -> Gain63/1, Zero-Order Hold20/1, Scope45/1
  Constant18/1 -> Sum52/1
  PID Controller1/1 -> Sum49/1
  Gain63/1 -> Sum49/2
  Sum52/1 -> PID Controller1/1
  Gain65/1 -> Integrator17/1
  Sum50/1 -> Gain65/1
  Gain66/1 -> Sum50/2
  PID Controller2/1 -> Scope46/2, Sum50/1
  Sum51/1 -> PID Controller2/1
  Integrator17/1 -> Scope46/1, Zero-Order Hold21/1, Gain66/1
  Step7/1 -> Sum51/1
  Step8/1 -> Scope70/2, Sum53/1
  Sum53/1 -> Scope55/2, PID Controller3/1
  PID Controller3/1 -> Scope55/1, Sum54/1
  Sum54/1 -> Goto18/1, Zero-Order Hold10/1
  Sum55/1 -> Sum47/2
  Random Source/1 -> Sum55/1
  Sum56/1 -> Sum54/2
  Random Source1/1 -> Sum56/1
  Zero-Order Hold10/1 -> Sum42/1
  Zero-Order Hold11/1 -> Sum44/1
  Zero-Order Hold13/1 -> Goto25/1, Sum61/1
  Random Source3/1 -> ?
  Sum58/1 -> Sum57/1
  From34/1 -> Product13/2
  MATLAB Function11/2(X_b) -> Scope51/2
  Product12/1 -> Gain78/1
  Gain68/1 -> Sum57/2
  Sin8/1 -> Gain72/1
  From35/1 -> MATLAB Function12/3(theta_e), MATLAB Function11/3(theta_e)
  Gain75/1 -> Integrator20/1
  MATLAB Function11/1(X_a) -> Scope51/1
  Gain73/1 -> Sin8/1
  Sum57/1 -> Gain67/1
  Sum62/1 -> Sum60/1
  Step9/1 -> Sum58/1
  Gain77/1 -> Integrator21/1
  Gain71/1 -> Goto23/1
  Integrator20/1 -> Gain74/1, Gain76/1, Goto21/1
  Sum59/1 -> Gain75/1
  Gain74/1 -> Sum58/2
  Sum61/1 -> Gain77/1
  From32/1 -> Product12/1, Gain79/1
  Gain76/1 -> Sum60/2
  Product13/1 -> Gain70/1
  MATLAB Function12/1(X_a) -> Scope50/1
  From37/1 -> Scope52/2, MATLAB Function11/2(X_d)
  Gain69/1 -> Sum63/2
  Zero-Order Hold12/1 -> Goto24/1, Sum59/1
  From36/1 -> MATLAB Function11/1(X_q), Scope52/1
  Integrator21/1 -> Gain69/1, Product12/2, Goto20/1
  From33/1 -> Product13/1
  Integrator19/1 -> Scope48/1, Gain68/1, Goto22/1, Integrator18/1
  MATLAB Function12/2(X_b) -> Scope50/2
  Gain70/1 -> Sum63/1
  Gain67/1 -> Integrator19/1
  Gain72/1 -> Sum58/3
  Gain79/1 -> Sum62/1
  FCS MPC/2(Vd) -> Zero-Order Hold13/1
  Sum60/1 -> Sum59/2
  Integrator18/1 -> Scope48/2, Gain71/1, Gain73/1
  From31/1 -> MATLAB Function12/1(X_q), Scope49/1
  From30/1 -> MATLAB Function12/2(X_d), Scope49/2
  Sum63/1 -> Sum61/2
  Gain78/1 -> Sum62/2
  Random Source2/1 -> ?
  FCS MPC/1(Vq) -> Zero-Order Hold12/1
  Constant19/1 -> To Workspace3/1, Scope54/2, Zero-Order Hold15/1
  Constant20/1 -> FCS MPC/7(Vcc)
  Constant21/1 -> FCS MPC/8(Ts)
  Zero-Order Hold14/1 -> FCS MPC/1(iq_ref)
  Zero-Order Hold15/1 -> FCS MPC/2(id_ref)
  From40/1 -> Zero-Order Hold18/1
  Zero-Order Hold18/1 -> FCS MPC/5(omega_m)
  Zero-Order Hold19/1 -> FCS MPC/6(theta_e)
  From41/1 -> Zero-Order Hold19/1
  Step10/1 -> Scope53/2, Zero-Order Hold14/1
  Zero-Order Hold20/1 -> Sum52/2
  Zero-Order Hold21/1 -> Sum51/2
  Zero-Order Hold22/1 -> Sum53/2
  Zero-Order Hold23/1 -> Sum48/2
  From44/1 -> Zero-Order Hold22/1
  PID Controller5/1 -> Sum74/1
  Sum73/1 -> PID Controller5/1
  PID Controller6/1 -> Sum71/1
  Sum72/1 -> PID Controller6/1
  Sum74/1 -> Goto30/1, Zero-Order Hold24/1
  Sum76/1 -> Sum74/2
  Sum75/1 -> Sum71/2
  Sum65/1 -> Sum64/1
  From49/1 -> Product15/2
  MATLAB Function13/2(X_b) -> Scope59/2
  Product14/1 -> Gain91/1
  Gain81/1 -> Sum64/2
  Sin9/1 -> Gain85/1
  From50/1 -> MATLAB Function14/3(theta_e), MATLAB Function13/3(theta_e)
  Gain88/1 -> Integrator24/1
  MATLAB Function13/1(X_a) -> Scope59/1
  Gain86/1 -> Sin9/1
  Sum64/1 -> Gain80/1
  Sum69/1 -> Sum67/1, Sum76/2
  Step11/1 -> Sum65/1
  Gain90/1 -> Integrator25/1
  Gain84/1 -> Goto29/1
  Integrator24/1 -> Gain87/1, Gain89/1, Goto27/1
  Sum66/1 -> Gain88/1
  Gain87/1 -> Sum65/2
  Sum68/1 -> Gain90/1
  From47/1 -> Product14/1, Gain92/1
  Gain89/1 -> Sum67/2
  Product15/1 -> Gain83/1
  MATLAB Function14/1(X_a) -> Scope58/1
  From52/1 -> Scope60/2, MATLAB Function13/2(X_d)
  Gain82/1 -> Sum70/2
  From51/1 -> MATLAB Function13/1(X_q), Scope60/1
  From48/1 -> Product15/1
  Constant22/1 -> Sum72/1
  Integrator23/1 -> Scope56/1, Gain81/1, Goto28/1, Integrator22/1
  MATLAB Function14/2(X_b) -> Scope58/2
  Gain83/1 -> Sum75/2, Sum70/1
  Gain80/1 -> Integrator23/1
  Gain85/1 -> Sum65/3
  Gain92/1 -> Sum69/1
  Sum71/1 -> Goto31/1, Zero-Order Hold25/1
  Sum67/1 -> Sum66/2
  Integrator22/1 -> Scope56/2, Gain84/1, Gain86/1
  From46/1 -> MATLAB Function14/1(X_q), Scope57/1
  From45/1 -> MATLAB Function14/2(X_d), Scope57/2
  Sum70/1 -> Sum68/2
  Gain91/1 -> Sum69/2
  Zero-Order Hold24/1 -> MATLAB Function15/1(X_q)
  Zero-Order Hold25/1 -> MATLAB Function15/2(X_d)
  MATLAB Function17/1(X_q) -> Sum66/1
  MATLAB Function17/2(X_d) -> Sum68/1
  From54/1 -> MATLAB Function17/3(theta_e)
  From55/1 -> MATLAB Function15/3(theta_e)
  MATLAB Function15/1(X_a) -> Modulator/1(u_a*)
  MATLAB Function15/2(X_b) -> Modulator/2(u_b*)
  Modulator/1(u_a) -> MATLAB Function17/1(X_a)
  Modulator/2(u_b) -> MATLAB Function17/2(X_b)
  Sum81/1 -> Gain103/1
  Zero-Order Hold30/1 -> Deadbeat Control/1(iq_ref)
  [i_q] -> Product17/2
  Gain99/1 -> Sin10/1
  Zero-Order Hold33/1 -> Deadbeat Control/4(id)
  Integrator26/1 -> Scope62/2, Gain97/1, Gain99/1
  [u_d] -> Scope66/2, MATLAB Function18/2(X_d)
  Sum77/1 -> Gain93/1
  Product17/1 -> Gain96/1
  MATLAB Function21/1(X_q) -> Sum79/1, [u_q]
  Gain98/1 -> Sum78/3
  Gain94/1 -> Sum77/2
  Constant23/1 -> Scope68/2, Zero-Order Hold31/1
  Gain95/1 -> Sum83/2
  [w_m] -> Product17/1
  Step13/1 -> Scope67/2, Zero-Order Hold30/1
  Sum82/1 -> Sum80/1
  [i_d] -> To Workspace/1, Scope68/1
  [i_q] -> Scope67/1
  Zero-Order Hold35/1 -> Deadbeat Control/6(theta_e)
  Zero-Order Hold31/1 -> Deadbeat Control/2(id_ref)
  Gain102/1 -> Sum80/2
  Zero-Order Hold34/1 -> Deadbeat Control/5(omega_m)
  Sum83/1 -> Sum81/2
  MATLAB Function19/1(X_a) -> Scope64/1
  Integrator27/1 -> Scope62/1, Gain94/1, [w_m], Integrator26/1
  Integrator28/1 -> Gain100/1, Gain102/1, [i_q]
  Sum79/1 -> Gain101/1
  Gain97/1 -> [theta_e]
  [u_q] -> MATLAB Function18/1(X_q), Scope66/1
  [theta_e] -> Zero-Order Hold35/1
  Gain104/1 -> Sum82/2
  [theta_e] -> MATLAB Function19/3(theta_e), MATLAB Function18/3(theta_e)
  MATLAB Function19/2(X_b) -> Scope64/2
  Gain103/1 -> Integrator29/1
  Gain96/1 -> Sum83/1
  Gain101/1 -> Integrator28/1
  Product16/1 -> Gain104/1
  Sum78/1 -> Sum77/1
  Zero-Order Hold32/1 -> Deadbeat Control/3(iq)
  MATLAB Function18/2(X_b) -> Scope65/2
  [w_m] -> Zero-Order Hold34/1
  MATLAB Function21/2(X_d) -> [u_d], Sum81/1
  Gain100/1 -> Sum78/2
  Constant24/1 -> Deadbeat Control/7(Vcc)
  Gain93/1 -> Integrator27/1
  Sum80/1 -> Sum79/2
  [i_d] -> MATLAB Function19/2(X_d), Scope63/2
  Step14/1 -> Sum78/1
  Integrator29/1 -> Gain95/1, Product16/2, [i_d]
  Gain105/1 -> Sum82/1
  Sin10/1 -> Gain98/1
  [w_m] -> Product16/1, Gain105/1
  MATLAB Function18/1(X_a) -> Scope65/1
  [i_q] -> MATLAB Function19/1(X_q), Scope63/1
  Constant25/1 -> Deadbeat Control/8(Ts)
  [theta_e] -> MATLAB Function21/3(theta_e)
  Modulator1/1(u_a) -> MATLAB Function21/1(X_a)
  [theta_e] -> MATLAB Function20/3(theta_e)
  Modulator1/2(u_b) -> MATLAB Function21/2(X_b)
  MATLAB Function20/2(X_b) -> Modulator1/2(u_b*)
  MATLAB Function20/1(X_a) -> Modulator1/1(u_a*)
  Deadbeat Control/1(Vq) -> Scope69/1, MATLAB Function20/1(X_q)
  Deadbeat Control/2(Vd) -> Scope69/2, MATLAB Function20/2(X_d)
  MATLAB Function5/1(X_d) -> Subsystem/1(u_d)
  MATLAB Function5/2(X_q) -> Subsystem/2(u_q)
  Subsystem/2(Out1) -> Gain12/1
  From2/1 -> Scope70/1
  Random Source6/1 -> ?
  Random Source7/1 -> ?
  Random Source8/1 -> Sum/2
  Sum/1 -> Zero-Order Hold32/1
  [i_q] -> Sum/1
  [i_d] -> Sum1/1
  Sum1/1 -> Zero-Order Hold33/1
  Random Source9/1 -> Sum1/2
  Random Source11/1 -> Sum3/2
  Random Source10/1 -> Sum2/2
  Sum3/1 -> To Workspace2/1, Scope54/1, Zero-Order Hold17/1
  From3/1 -> Sum2/1
  From4/1 -> Sum3/1
  Zero-Order Hold16/1 -> FCS MPC/3(iq)
  Zero-Order Hold17/1 -> FCS MPC/4(id)
  From76/1 -> Sum4/1
  Integrator3/1 -> Gain1/1, Gain3/1, Goto2/1
  MATLAB Function25/2(X_d) -> Sum87/1, Goto38/1
  From42/1 -> Product1/1, Gain6/1
  Gain4/1 -> Integrator30/1
  From83/1 -> MATLAB Function24/3(theta_e)
  From43/1 -> Product18/1
  Constant27/1 -> Deadbeat Control1/7(Vcc)
  Sum84/1 -> Sum6/1
  Constant28/1 -> Deadbeat Control1/8(Ts)
  Random Source15/1 -> Sum5/2
  MATLAB Function24/2(X_b) -> Modulator2/2(u_b*)
  Sum86/1 -> Sum85/2
  Sum4/1 -> Zero-Order Hold36/1
  Zero-Order Hold38/1 -> Deadbeat Control1/5(omega_m)
  Gain13/1 -> Sum84/3
  Gain6/1 -> Sum88/1
  Random Source14/1 -> Sum4/2
  Gain8/1 -> Sum6/2
  From79/1 -> Zero-Order Hold39/1
  Modulator2/2(u_b) -> MATLAB Function25/2(X_b)
  Sin11/1 -> Gain13/1
  Deadbeat Control1/1(Vq) -> MATLAB Function24/1(X_q)
  MATLAB Function24/1(X_a) -> Modulator2/1(u_a*)
  Sum89/1 -> Sum87/2
  Gain3/1 -> Sum86/2
  From82/1 -> MATLAB Function25/3(theta_e)
  Integrator30/1 -> Gain9/1, Product1/2, Goto1/1
  Step16/1 -> Sum84/1
  Gain1/1 -> Sum84/2
  From78/1 -> Zero-Order Hold38/1
  Gain2/1 -> Integrator3/1
  Sum85/1 -> Gain2/1
  Modulator2/1(u_a) -> MATLAB Function25/1(X_a)
  Gain7/1 -> Integrator2/1
  Gain10/1 -> Sum89/1
  Gain5/1 -> Sum88/2
  Constant26/1 -> Zero-Order Hold29/1
  Deadbeat Control1/2(Vd) -> MATLAB Function24/2(X_d)
  Sum88/1 -> Sum86/1
  Gain11/1 -> Goto6/1
  Gain106/1 -> Sin11/1
  Sum5/1 -> Zero-Order Hold37/1
  Zero-Order Hold29/1 -> Deadbeat Control1/2(id_ref)
  Zero-Order Hold39/1 -> Deadbeat Control1/6(theta_e)
  From72/1 -> Product18/2
  Integrator2/1 -> Gain8/1, Goto3/1, Integrator1/1
  Product1/1 -> Gain5/1
  Step15/1 -> Zero-Order Hold28/1
  Gain9/1 -> Sum89/2
  Zero-Order Hold36/1 -> Deadbeat Control1/3(iq)
  MATLAB Function25/1(X_q) -> Goto7/1, Sum85/1
  Product18/1 -> Gain10/1
  Sum6/1 -> Gain7/1
  Integrator1/1 -> Gain106/1, Gain11/1
  Sum87/1 -> Gain4/1
  Zero-Order Hold28/1 -> Deadbeat Control1/1(iq_ref)
  Zero-Order Hold37/1 -> Deadbeat Control1/4(id)
  From77/1 -> Sum5/1
  Random Source16/1 -> ?
  Random Source17/1 -> ?
  Random Source12/1 -> Sum90/2
  Zero-Order Hold45/1 -> FCS MPC1/4(id)
  Zero-Order Hold44/1 -> FCS MPC1/3(iq)
  From38/1 -> Sum90/1
  From86/1 -> Sum91/1
  Sum90/1 -> Zero-Order Hold44/1
  Sum91/1 -> Zero-Order Hold45/1
  Random Source13/1 -> Sum91/2
  Zero-Order Hold40/1 -> Goto43/1, Sum94/1
  Integrator31/1 -> Gain111/1, Gain113/1
  Integrator32/1 -> Gain108/1, Goto41/1, Integrator31/1
  Sin12/1 -> Gain112/1
  Sum95/1 -> Sum94/2
  From74/1 -> Product19/1, Gain119/1
  Gain111/1 -> Goto42/1
  Sum97/1 -> Sum95/1
  Zero-Order Hold47/1 -> FCS MPC1/6(theta_e)
  Gain113/1 -> Sin12/1
  Zero-Order Hold42/1 -> FCS MPC1/1(iq_ref)
  From80/1 -> Product20/2
  Gain112/1 -> Sum93/3
  From88/1 -> Zero-Order Hold47/1
  Step17/1 -> Zero-Order Hold42/1
  Constant30/1 -> FCS MPC1/7(Vcc)
  Constant29/1 -> Zero-Order Hold43/1
  Constant31/1 -> FCS MPC1/8(Ts)
  Gain118/1 -> Sum97/2
  Sum98/1 -> Sum96/2
  Integrator33/1 -> Gain114/1, Gain116/1, Goto40/1
  Integrator34/1 -> Gain109/1, Product19/2, Goto39/1
  FCS MPC1/2(Vd) -> Zero-Order Hold41/1
  Gain119/1 -> Sum97/1
  Sum92/1 -> Gain107/1
  FCS MPC1/1(Vq) -> Zero-Order Hold40/1
  Zero-Order Hold43/1 -> FCS MPC1/2(id_ref)
  Sum93/1 -> Sum92/1
  From75/1 -> Product20/1
  Gain107/1 -> Integrator32/1
  From87/1 -> Zero-Order Hold46/1
  Gain110/1 -> Sum98/1
  Gain116/1 -> Sum95/2
  Gain117/1 -> Integrator34/1
  Gain109/1 -> Sum98/2
  Sum94/1 -> Gain115/1
  Step18/1 -> Sum93/1
  Gain114/1 -> Sum93/2
  Zero-Order Hold46/1 -> FCS MPC1/5(omega_m)
  Product20/1 -> Gain110/1
  Sum96/1 -> Gain117/1
  Product19/1 -> Gain118/1
  Gain108/1 -> Sum92/2
  Gain115/1 -> Integrator33/1
  Zero-Order Hold41/1 -> Goto44/1, Sum96/1
  Sum2/1 -> Zero-Order Hold16/1, Scope53/1
  Zero-Order Hold26/1 -> Sum99/2
  Sum99/1 -> Sum73/2
  ? -> Sum99/1
  Random Source18/1 -> Sum100/1
  Zero-Order Hold27/1 -> Sum100/2
  Sum100/1 -> Sum72/2
  Step12/1 -> To Workspace5/1, Scope61/1, Sum73/1
  From53/1 -> To Workspace4/1, Scope61/2, Zero-Order Hold26/1
  Integrator25/1 -> Gain82/1, Zero-Order Hold27/1, To Workspace6/1, Product14/2, Goto26/1
  connections:
  DC Voltage Source/RConn1 -- Full-Bridge Converter/RConn1
  Full-Bridge Converter/RConn2 -- DC Voltage Source/LConn1
  Stepper Motor/LConn4 -- Full-Bridge Converter/LConn1
  Stepper Motor/LConn3 -- Full-Bridge Converter/LConn2
  Inductor/LConn1 -- Voltage Source/LConn1 -- Voltage Sensor/LConn1
  Inductor/RConn1 -- Resistor/LConn1
  Electrical Reference1/LConn1 -- Voltage Source/RConn1 -- Controlled Voltage Source/LConn1 -- Voltage Sensor/RConn2
  Current Sensor/LConn1 -- Resistor/RConn1
  Controlled Voltage Source/RConn2 -- Current Sensor/RConn2
  PS Math Function1/RConn1 -- PS Product/LConn1 -- PS Product2/LConn2
  Inductor1/LConn1 -- Voltage Sensor1/LConn1 -- Voltage Source1/LConn1
  PS Product1/LConn2 -- Current Sensor1/RConn1 -- PS-Simulink Converter5/LConn1
  PS Math Function2/RConn1 -- PS Product3/LConn2 -- PS Product1/LConn1
  Current Sensor1/LConn1 -- Resistor1/RConn1
  Inductor1/RConn1 -- Resistor1/LConn1
  Current Sensor1/RConn2 -- Controlled Voltage Source1/LConn1
  Electrical Reference/LConn1 -- Controlled Voltage Source1/RConn2 -- Voltage Sensor1/RConn2 -- Voltage Source1/RConn1 -- Solver Configuration/RConn1
  PS Product1/RConn1 -- PS Add/LConn2
  PS Product/RConn1 -- PS Add/LConn1
  PS Gain/RConn1 -- PS Product/LConn2
  PS Gain/LConn1 -- PS-Simulink Converter4/LConn1 -- Current Sensor/RConn1
  PS Gain1/LConn1 -- PS Add/RConn1
  Inertia/LConn1 -- Rotational Damper/LConn1 -- Ideal Rotational Motion Sensor/LConn1 -- Ideal Torque Source2/LConn1 -- Ideal Torque Source/LConn1 -- Ideal Torque Source1/LConn1
  Rotational Damper/RConn1 -- Mechanical Rotational Reference/LConn1
  Simulink-PS Converter/RConn1 -- Ideal Torque Source1/RConn1
  Mechanical Rotational Reference1/LConn1 -- Ideal Torque Source/RConn2 -- Ideal Torque Source2/RConn2
  Mechanical Rotational Reference2/LConn1 -- Ideal Rotational Motion Sensor/RConn1 -- Ideal Torque Source1/RConn2
  Ideal Rotational Motion Sensor/RConn2 -- PS-Simulink Converter2/LConn1 -- PS Gain5/LConn1 -- PS-Simulink Converter/LConn1
  Ideal Rotational Motion Sensor/RConn3 -- PS-Simulink Converter3/LConn1 -- PS Gain2/LConn1 -- PS Gain4/LConn1 -- PS-Simulink Converter1/LConn1
  PS Math Function3/LConn1 -- PS Gain2/RConn1
  PS Gain3/LConn1 -- PS Math Function3/RConn1
  PS Gain3/RConn1 -- Ideal Torque Source2/RConn1
  PS Gain4/RConn1 -- PS Math Function2/LConn1 -- PS Math Function1/LConn1
  PS Gain1/RConn1 -- PS-Simulink Converter6/LConn1 -- Ideal Torque Source/RConn1
  PS Product2/RConn1 -- Controlled Voltage Source/RConn1
  PS Gain5/RConn1 -- PS Product2/LConn1 -- PS Product3/LConn1
  Controlled Voltage Source1/RConn1 -- PS Product3/RConn1
  Controlled PWM Voltage/RConn1 -- Voltage Sensor3/LConn1 -- H-Bridge2/LConn1
  Voltage Source2/LConn1 -- Voltage Sensor2/LConn1 -- Controlled PWM Voltage/LConn1
  Voltage Source2/RConn1 -- Controlled PWM Voltage/LConn2 -- Electrical Reference4/LConn1
  H-Bridge2/RConn4 -- Electrical Reference2/LConn1
  Voltage Source3/LConn1 -- H-Bridge2/RConn1
  Electrical Reference3/LConn1 -- Solver Configuration1/RConn1 -- Voltage Source3/RConn1
  Electrical Reference5/LConn1 -- H-Bridge2/LConn4 -- H-Bridge2/LConn3 -- H-Bridge2/LConn2 -- Controlled PWM Voltage/RConn2
  PS-Simulink Converter10/LConn1 -- Voltage Sensor2/RConn1
  Electrical Reference6/LConn1 -- Voltage Sensor3/RConn2
  Voltage Sensor3/RConn1 -- PS-Simulink Converter11/LConn1
  Electrical Reference7/LConn1 -- Voltage Sensor2/RConn2
  Voltage Sensor4/RConn2 -- Resistor2/RConn1 -- Ideal Semiconductor Switch1/RConn1 -- Ideal Semiconductor Switch/RConn2 -- Half-Bridge Driver/RConn2
  Ideal Semiconductor Switch1/LConn1 -- Half-Bridge Driver/RConn3
  Half-Bridge Driver/RConn4 -- Ideal Semiconductor Switch1/RConn2 -- Electrical Reference13/LConn1
  Half-Bridge Driver1/RConn2 -- Current Sensor2/LConn1 -- Voltage Sensor4/LConn1 -- Ideal Semiconductor Switch3/RConn2 -- Ideal Semiconductor Switch2/RConn1
  Ideal Semiconductor Switch3/LConn1 -- Half-Bridge Driver1/RConn1
  Ideal Semiconductor Switch2/LConn1 -- Half-Bridge Driver1/RConn3
  Half-Bridge Driver1/RConn4 -- Half-Bridge Driver1/LConn2 -- Ideal Semiconductor Switch2/RConn2 -- Electrical Reference14/LConn1
  Ideal Semiconductor Switch/LConn1 -- Half-Bridge Driver/RConn1
  Controlled PWM Voltage1/LConn1 -- Voltage Source4/LConn1 -- Voltage Sensor5/LConn1
  Electrical Reference8/LConn1 -- Solver Configuration2/RConn1 -- Voltage Source5/RConn1
  Electrical Reference9/LConn1 -- Controlled PWM Voltage1/LConn2 -- Voltage Source4/RConn1
  Electrical Reference11/LConn1 -- Voltage Sensor5/RConn2
  Electrical Reference10/LConn1 -- Voltage Sensor6/RConn2
  CMOS NOT/LConn1 -- Half-Bridge Driver/LConn1 -- Controlled PWM Voltage1/RConn1 -- Voltage Sensor6/LConn1
  Controlled PWM Voltage1/RConn2 -- Half-Bridge Driver/LConn2 -- Electrical Reference12/LConn1
  Voltage Source5/LConn1 -- Ideal Semiconductor Switch3/RConn1 -- Ideal Semiconductor Switch/RConn1
  Current Sensor2/RConn1 -- PS-Simulink Converter8/LConn1
  CMOS NOT/RConn1 -- Half-Bridge Driver1/LConn1
  Voltage Sensor6/RConn1 -- PS-Simulink Converter12/LConn1
  Voltage Sensor5/RConn1 -- PS-Simulink Converter13/LConn1
  Inductor2/RConn1 -- Resistor2/LConn1
  Voltage Sensor4/RConn1 -- PS-Simulink Converter9/LConn1
  Inductor2/LConn1 -- Current Sensor2/RConn2
  Ideal Semiconductor Switch4/LConn1 -- Half-Bridge Driver2/RConn1
  Ideal Semiconductor Switch5/LConn1 -- Half-Bridge Driver2/RConn3
  Ideal Semiconductor Switch6/LConn1 -- Half-Bridge Driver3/RConn1
  Ideal Semiconductor Switch7/LConn1 -- Half-Bridge Driver3/RConn3
  Ideal Semiconductor Switch8/LConn1 -- Half-Bridge Driver4/RConn1
  Ideal Semiconductor Switch9/LConn1 -- Half-Bridge Driver4/RConn3
  Ideal Semiconductor Switch10/LConn1 -- Half-Bridge Driver5/RConn1
  Ideal Semiconductor Switch11/LConn1 -- Half-Bridge Driver5/RConn3
  Electrical Reference15/LConn1 -- Half-Bridge Driver2/RConn4 -- Ideal Semiconductor Switch5/RConn2
  Ideal Semiconductor Switch5/RConn1 -- Ideal Semiconductor Switch4/RConn2 -- Half-Bridge Driver2/RConn2 -- Voltage Sensor7/LConn1 -- Inductor3/LConn1
  Electrical Reference16/LConn1 -- Half-Bridge Driver3/RConn4 -- Ideal Semiconductor Switch7/RConn2
  Ideal Semiconductor Switch7/RConn1 -- Ideal Semiconductor Switch6/RConn2 -- Half-Bridge Driver3/RConn2 -- Voltage Sensor7/RConn2 -- Current Sensor3/RConn2
  Electrical Reference17/LConn1 -- Half-Bridge Driver4/RConn4 -- Ideal Semiconductor Switch9/RConn2
  Ideal Semiconductor Switch9/RConn1 -- Ideal Semiconductor Switch8/RConn2 -- Half-Bridge Driver4/RConn2 -- Inductor4/LConn1
  Ideal Semiconductor Switch11/RConn2 -- Electrical Reference18/LConn1 -- Half-Bridge Driver5/RConn4
  Ideal Semiconductor Switch11/RConn1 -- Half-Bridge Driver5/RConn2 -- Ideal Semiconductor Switch10/RConn2 -- Resistor6/RConn1
  Voltage Source6/RConn1 -- Electrical Reference19/LConn1 -- Solver Configuration3/RConn1
  Voltage Source6/LConn1 -- Ideal Semiconductor Switch10/RConn1 -- Ideal Semiconductor Switch8/RConn1 -- Ideal Semiconductor Switch6/RConn1 -- Ideal Semiconductor Switch4/RConn1
  Inductor3/RConn1 -- Resistor5/LConn1
  Inductor4/RConn1 -- Resistor6/LConn1
  Voltage Sensor7/RConn1 -- PS-Simulink Converter7/LConn1
  Resistor5/RConn1 -- Current Sensor3/LConn1
  Current Sensor3/RConn1 -- PS-Simulink Converter14/LConn1
  Half-Bridge Driver3/LConn1 -- Simulink-PS Converter2/RConn1
  Simulink-PS Converter1/RConn1 -- Half-Bridge Driver2/LConn1
  Simulink-PS Converter3/RConn1 -- Half-Bridge Driver4/LConn1
  Simulink-PS Converter4/RConn1 -- Half-Bridge Driver5/LConn1
  PS Product7/LConn1 -- PS Gain11/RConn1 -- PS Product6/LConn1
  Ideal Torque Source3/RConn1 -- PS Gain7/RConn1 -- PS-Simulink Converter21/LConn1
  PS Math Function4/LConn1 -- PS Gain10/RConn1 -- PS Math Function5/LConn1
  PS-Simulink Converter16/LConn1 -- PS Gain8/LConn1 -- PS Gain10/LConn1 -- Ideal Rotational Motion Sensor1/RConn3 -- PS-Simulink Converter18/LConn1
  PS-Simulink Converter20/LConn1 -- PS Product5/LConn2 -- Current Sensor5/RConn1
  Ideal Torque Source5/RConn2 -- Mechanical Rotational Reference4/LConn1 -- Ideal Torque Source3/RConn2
  PS Product6/LConn2 -- PS Math Function4/RConn1 -- PS Product4/LConn1
  PS-Simulink Converter15/LConn1 -- Ideal Rotational Motion Sensor1/RConn2 -- PS-Simulink Converter17/LConn1 -- PS Gain11/LConn1
  Voltage Source8/LConn1 -- Inductor6/LConn1 -- Voltage Sensor9/LConn1
  Ideal Torque Source4/LConn1 -- Inertia1/LConn1 -- Rotational Damper1/LConn1 -- Ideal Rotational Motion Sensor1/LConn1 -- Ideal Torque Source5/LConn1 -- Ideal Torque Source3/LConn1
  Voltage Source8/RConn1 -- Electrical Reference20/LConn1 -- Solver Configuration4/RConn1 -- Controlled Voltage Source3/RConn2 -- Voltage Sensor9/RConn2
  Current Sensor4/RConn1 -- PS Gain6/LConn1 -- PS-Simulink Converter19/LConn1
  Controlled Voltage Source2/LConn1 -- Electrical Reference21/LConn1 -- Voltage Sensor8/RConn2 -- Voltage Source7/RConn1
  PS Product5/LConn1 -- PS Math Function5/RConn1 -- PS Product7/LConn2
  Voltage Sensor8/LConn1 -- Inductor5/LConn1 -- Voltage Source7/LConn1
  Ideal Torque Source4/RConn2 -- Mechanical Rotational Reference5/LConn1 -- Ideal Rotational Motion Sensor1/RConn1
  Inductor5/RConn1 -- Resistor7/LConn1
  Inductor6/RConn1 -- Resistor8/LConn1
  PS Product5/RConn1 -- PS Add1/LConn2
  PS Math Function6/LConn1 -- PS Gain8/RConn1
  PS Gain9/RConn1 -- Ideal Torque Source5/RConn1
  Controlled Voltage Source3/RConn1 -- PS Product7/RConn1
  Rotational Damper1/RConn1 -- Mechanical Rotational Reference3/LConn1
  Current Sensor4/LConn1 -- Resistor7/RConn1
  Current Sensor5/LConn1 -- Resistor8/RConn1
  Controlled Voltage Source2/RConn2 -- Current Sensor4/RConn2
  PS Product6/RConn1 -- Controlled Voltage Source2/RConn1
  PS Gain9/LConn1 -- PS Math Function6/RConn1
  Current Sensor5/RConn2 -- Controlled Voltage Source3/LConn1
  PS Gain7/LConn1 -- PS Add1/RConn1
  PS Gain6/RConn1 -- PS Product4/LConn2
  Simulink-PS Converter5/RConn1 -- Ideal Torque Source4/RConn1
  PS Product4/RConn1 -- PS Add1/LConn1
